simulink model "UR5_OpenLoop"  (R2023b)
settings: Solver=FixedStepAuto  StartTime=0.0  StopTime=t_max  FixedStep=dt_max  RelTol=1e-3
values from neighbouring files (symbols this model uses):
  dt_max = 0.01    [UR5_Details.m]    (also in mpc_script.m; smc.m)
(part 2 of 2)

== matlab function UR5_OpenLoop/UR5 Kineamatics and Dynamics ==
  data: q_1 input; q_2 input; q_3 input; T output; Jacobi output; M output; C output; G output; dq_1 input; dq_2 input; dq_3 input; g parameter
function [T,Jacobi, M,C,G]    = fwdKIN(q_1, q_2, q_3, dq_1, dq_2,dq_3, g)

% TRANSLATION MATRICES AND FORWARD KINEMATICS 
% (Position of EE from joint space)
T = [cos(q_1)*cos(q_2)*cos(q_3) - 1.0*cos(q_1)*sin(q_2)*sin(q_3), - 1.0*cos(q_1)*cos(q_2)*sin(q_3) - 1.0*cos(q_1)*cos(q_3)*sin(q_2),  1.0*sin(q_1), 0.425*cos(q_1)*cos(q_2);
cos(q_2)*cos(q_3)*sin(q_1) - 1.0*sin(q_1)*sin(q_2)*sin(q_3), - 1.0*cos(q_2)*sin(q_1)*sin(q_3) - 1.0*cos(q_3)*sin(q_1)*sin(q_2), -1.0*cos(q_1), 0.425*cos(q_2)*sin(q_1);
              1.0*cos(q_2)*sin(q_3) + 1.0*cos(q_3)*sin(q_2),                     1.0*cos(q_2)*cos(q_3) - 1.0*sin(q_2)*sin(q_3),             0, 0.425*sin(q_2) + 0.0892;
                                                          0,                                                                 0,             0,                     1.0];
 

% JACOBIAN MATRIX OF END EFFECTOR
Jacobi = [0.0265*cos(q_1) + 1.0*sin(q_1)*(0.2723*sin(q_2)*sin(q_3) - 1.0*cos(q_2)*(0.2723*cos(q_3) + 0.425)), -1.0*cos(q_1)*(0.2723*cos(q_2)*sin(q_3) + 1.0*sin(q_2)*(0.2723*cos(q_3) + 0.425)), -1.0*cos(q_1)*(0.2723*cos(q_2)*sin(q_3) + 0.2723*cos(q_3)*sin(q_2));
0.0265*sin(q_1) - 1.0*cos(q_1)*(0.2723*sin(q_2)*sin(q_3) - 1.0*cos(q_2)*(0.2723*cos(q_3) + 0.425)), -1.0*sin(q_1)*(0.2723*cos(q_2)*sin(q_3) + 1.0*sin(q_2)*(0.2723*cos(q_3) + 0.425)), -1.0*sin(q_1)*(0.2723*cos(q_2)*sin(q_3) + 0.2723*cos(q_3)*sin(q_2));
                                                                                                 0,                 1.0*cos(q_2)*(0.2723*cos(q_3) + 0.425) - 0.2723*sin(q_2)*sin(q_3),                 0.2723*cos(q_2)*cos(q_3) - 0.2723*sin(q_2)*sin(q_3);
                                                                                                 0,                                                                      1.0*sin(q_1),                                                        1.0*sin(q_1);
                                                                                                 0,                                                                     -1.0*cos(q_1),                                                       -1.0*cos(q_1);
                                                                                               1.0,                                                                                 0,                                                                   0];


%Robots Inertia (Mass Matrix)
M = [                                                 1.378e-5*cos(q_1)^2 + 0.0021*cos(q_2)^2 + 1.378e-5*sin(q_1)^2 + 0.0078*sin(q_2)^2 + (0.1134*cos(q_1) - 0.2125*cos(q_2)*sin(q_1))*(0.9514*cos(q_1) - 1.784*cos(q_2)*sin(q_1)) + (0.1134*sin(q_1) + 0.2125*cos(q_1)*cos(q_2))*(0.9514*sin(q_1) + 1.784*cos(q_1)*cos(q_2)) + (0.0265*cos(q_1) + 1.0*sin(q_1)*(0.2723*sin(q_2)*sin(q_3) - 1.0*cos(q_2)*(0.2723*cos(q_3) + 0.425)))*(0.06029*cos(q_1) + 2.275*sin(q_1)*(0.2723*sin(q_2)*sin(q_3) - 1.0*cos(q_2)*(0.2723*cos(q_3) + 0.425))) + (0.0265*sin(q_1) - 1.0*cos(q_1)*(0.2723*sin(q_2)*sin(q_3) - 1.0*cos(q_2)*(0.2723*cos(q_3) + 0.425)))*(0.06029*sin(q_1) - 2.275*cos(q_1)*(0.2723*sin(q_2)*sin(q_3) - 1.0*cos(q_2)*(0.2723*cos(q_3) + 0.425))) + 1.0*(1.0*cos(q_2)*cos(q_3) - 1.0*sin(q_2)*sin(q_3))*(0.0462*cos(q_2)*cos(q_3) - 0.0462*sin(q_2)*sin(q_3)) + 1.0*(1.0*cos(q_2)*sin(q_3) + 1.0*cos(q_3)*sin(q_2))*(0.0016*cos(q_2)*sin(q_3) + 0.0016*cos(q_3)*sin(q_2)) + 0.0084,                                                                                                                                                                                                                                                                                                                                                                                                                                                                                                                                                                          1.0*sin(q_1)*((0.0016*cos(q_2)*sin(q_3) + 0.0016*cos(q_3)*sin(q_2))*(cos(q_1)*cos(q_2)*cos(q_3) - 1.0*cos(q_1)*sin(q_2)*sin(q_3)) - 1.0*(0.0462*cos(q_2)*cos(q_3) - 0.0462*sin(q_2)*sin(q_3))*(1.0*cos(q_1)*cos(q_2)*sin(q_3) + 1.0*cos(q_1)*cos(q_3)*sin(q_2))) + 1.0*cos(q_1)*((0.0462*cos(q_2)*cos(q_3) - 0.0462*sin(q_2)*sin(q_3))*(1.0*cos(q_2)*sin(q_1)*sin(q_3) + 1.0*cos(q_3)*sin(q_1)*sin(q_2)) + (0.0016*cos(q_2)*sin(q_3) + 0.0016*cos(q_3)*sin(q_2))*(1.0*sin(q_1)*sin(q_2)*sin(q_3) - 1.0*cos(q_2)*cos(q_3)*sin(q_1))) - 0.2125*cos(q_1)*sin(q_2)*(0.9514*cos(q_1) - 1.784*cos(q_2)*sin(q_1)) - 0.2125*sin(q_1)*sin(q_2)*(0.9514*sin(q_1) + 1.784*cos(q_1)*cos(q_2)) - 1.0*cos(q_1)*(0.06029*cos(q_1) + 2.275*sin(q_1)*(0.2723*sin(q_2)*sin(q_3) - 1.0*cos(q_2)*(0.2723*cos(q_3) + 0.425)))*(0.2723*cos(q_2)*sin(q_3) + 1.0*sin(q_2)*(0.2723*cos(q_3) + 0.425)) - 1.0*sin(q_1)*(0.06029*sin(q_1) - 2.275*cos(q_1)*(0.2723*sin(q_2)*sin(q_3) - 1.0*cos(q_2)*(0.2723*cos(q_3) + 0.425)))*(0.2723*cos(q_2)*sin(q_3) + 1.0*sin(q_2)*(0.2723*cos(q_3) + 0.425)),                                                                                                                                                                                                                                                                                                                                                                                                                                                                                                                                                                                                                                                 1.0*sin(q_1)*((0.0016*cos(q_2)*sin(q_3) + 0.0016*cos(q_3)*sin(q_2))*(cos(q_1)*cos(q_2)*cos(q_3) - 1.0*cos(q_1)*sin(q_2)*sin(q_3)) - 1.0*(0.0462*cos(q_2)*cos(q_3) - 0.0462*sin(q_2)*sin(q_3))*(1.0*cos(q_1)*cos(q_2)*sin(q_3) + 1.0*cos(q_1)*cos(q_3)*sin(q_2))) + 1.0*cos(q_1)*((0.0462*cos(q_2)*cos(q_3) - 0.0462*sin(q_2)*sin(q_3))*(1.0*cos(q_2)*sin(q_1)*sin(q_3) + 1.0*cos(q_3)*sin(q_1)*sin(q_2)) + (0.0016*cos(q_2)*sin(q_3) + 0.0016*cos(q_3)*sin(q_2))*(1.0*sin(q_1)*sin(q_2)*sin(q_3) - 1.0*cos(q_2)*cos(q_3)*sin(q_1))) - 1.0*cos(q_1)*(0.2723*cos(q_2)*sin(q_3) + 0.2723*cos(q_3)*sin(q_2))*(0.06029*cos(q_1) + 2.275*sin(q_1)*(0.2723*sin(q_2)*sin(q_3) - 1.0*cos(q_2)*(0.2723*cos(q_3) + 0.425))) - 1.0*sin(q_1)*(0.2723*cos(q_2)*sin(q_3) + 0.2723*cos(q_3)*sin(q_2))*(0.06029*sin(q_1) - 2.275*cos(q_1)*(0.2723*sin(q_2)*sin(q_3) - 1.0*cos(q_2)*(0.2723*cos(q_3) + 0.425)));
1.0*(1.0*cos(q_2)*sin(q_3) + 1.0*cos(q_3)*sin(q_2))*(0.0016*cos(q_1)*(1.0*sin(q_1)*sin(q_2)*sin(q_3) - 1.0*cos(q_2)*cos(q_3)*sin(q_1)) + 0.0016*sin(q_1)*(cos(q_1)*cos(q_2)*cos(q_3) - 1.0*cos(q_1)*sin(q_2)*sin(q_3))) + 1.0*(1.0*cos(q_2)*cos(q_3) - 1.0*sin(q_2)*sin(q_3))*(0.0462*cos(q_1)*(1.0*cos(q_2)*sin(q_1)*sin(q_3) + 1.0*cos(q_3)*sin(q_1)*sin(q_2)) - 0.0462*sin(q_1)*(1.0*cos(q_1)*cos(q_2)*sin(q_3) + 1.0*cos(q_1)*cos(q_3)*sin(q_2))) - 1.784*cos(q_1)*sin(q_2)*(0.1134*cos(q_1) - 0.2125*cos(q_2)*sin(q_1)) - 1.784*sin(q_1)*sin(q_2)*(0.1134*sin(q_1) + 0.2125*cos(q_1)*cos(q_2)) - 2.275*cos(q_1)*(0.0265*cos(q_1) + 1.0*sin(q_1)*(0.2723*sin(q_2)*sin(q_3) - 1.0*cos(q_2)*(0.2723*cos(q_3) + 0.425)))*(0.2723*cos(q_2)*sin(q_3) + 1.0*sin(q_2)*(0.2723*cos(q_3) + 0.425)) - 2.275*sin(q_1)*(0.0265*sin(q_1) - 1.0*cos(q_1)*(0.2723*sin(q_2)*sin(q_3) - 1.0*cos(q_2)*(0.2723*cos(q_3) + 0.425)))*(0.2723*cos(q_2)*sin(q_3) + 1.0*sin(q_2)*(0.2723*cos(q_3) + 0.425)), 0.379*cos(q_2)^2 + 2.275*cos(q_1)^2*(0.2723*cos(q_2)*sin(q_3) + 1.0*sin(q_2)*(0.2723*cos(q_3) + 0.425))^2 + (0.2723*sin(q_2)*sin(q_3) - 1.0*cos(q_2)*(0.2723*cos(q_3) + 0.425))*(0.6195*sin(q_2)*sin(q_3) - 2.275*cos(q_2)*(0.2723*cos(q_3) + 0.425)) + 2.275*sin(q_1)^2*(0.2723*cos(q_2)*sin(q_3) + 1.0*sin(q_2)*(0.2723*cos(q_3) + 0.425))^2 + 1.0*cos(q_1)^2*(0.0021*cos(q_1)^2 + 0.0021*sin(q_1)^2) + 1.0*sin(q_1)^2*(0.0021*cos(q_1)^2 + 0.0021*sin(q_1)^2) + 0.379*cos(q_1)^2*sin(q_2)^2 + 1.0*sin(q_1)*(1.0*sin(q_1)*(0.0462*cos(q_1)^2 + 0.0462*sin(q_1)^2) - 1.0*(0.0462*cos(q_1)*(1.0*cos(q_2)*sin(q_1)*sin(q_3) + 1.0*cos(q_3)*sin(q_1)*sin(q_2)) - 0.0462*sin(q_1)*(1.0*cos(q_1)*cos(q_2)*sin(q_3) + 1.0*cos(q_1)*cos(q_3)*sin(q_2)))*(1.0*cos(q_1)*cos(q_2)*sin(q_3) + 1.0*cos(q_1)*cos(q_3)*sin(q_2)) + (cos(q_1)*cos(q_2)*cos(q_3) - 1.0*cos(q_1)*sin(q_2)*sin(q_3))*(0.0016*cos(q_1)*(1.0*sin(q_1)*sin(q_2)*sin(q_3) - 1.0*cos(q_2)*cos(q_3)*sin(q_1)) + 0.0016*sin(q_1)*(cos(q_1)*cos(q_2)*cos(q_3) - 1.0*cos(q_1)*sin(q_2)*sin(q_3)))) + 0.379*sin(q_1)^2*sin(q_2)^2 + 1.0*cos(q_1)*((1.0*sin(q_1)*sin(q_2)*sin(q_3) - 1.0*cos(q_2)*cos(q_3)*sin(q_1))*(0.0016*cos(q_1)*(1.0*sin(q_1)*sin(q_2)*sin(q_3) - 1.0*cos(q_2)*cos(q_3)*sin(q_1)) + 0.0016*sin(q_1)*(cos(q_1)*cos(q_2)*cos(q_3) - 1.0*cos(q_1)*sin(q_2)*sin(q_3))) + (0.0462*cos(q_1)*(1.0*cos(q_2)*sin(q_1)*sin(q_3) + 1.0*cos(q_3)*sin(q_1)*sin(q_2)) - 0.0462*sin(q_1)*(1.0*cos(q_1)*cos(q_2)*sin(q_3) + 1.0*cos(q_1)*cos(q_3)*sin(q_2)))*(1.0*cos(q_2)*sin(q_1)*sin(q_3) + 1.0*cos(q_3)*sin(q_1)*sin(q_2)) + 1.0*cos(q_1)*(0.0462*cos(q_1)^2 + 0.0462*sin(q_1)^2)), 1.0*sin(q_1)*(1.0*sin(q_1)*(0.0462*cos(q_1)^2 + 0.0462*sin(q_1)^2) - 1.0*(0.0462*cos(q_1)*(1.0*cos(q_2)*sin(q_1)*sin(q_3) + 1.0*cos(q_3)*sin(q_1)*sin(q_2)) - 0.0462*sin(q_1)*(1.0*cos(q_1)*cos(q_2)*sin(q_3) + 1.0*cos(q_1)*cos(q_3)*sin(q_2)))*(1.0*cos(q_1)*cos(q_2)*sin(q_3) + 1.0*cos(q_1)*cos(q_3)*sin(q_2)) + (cos(q_1)*cos(q_2)*cos(q_3) - 1.0*cos(q_1)*sin(q_2)*sin(q_3))*(0.0016*cos(q_1)*(1.0*sin(q_1)*sin(q_2)*sin(q_3) - 1.0*cos(q_2)*cos(q_3)*sin(q_1)) + 0.0016*sin(q_1)*(cos(q_1)*cos(q_2)*cos(q_3) - 1.0*cos(q_1)*sin(q_2)*sin(q_3)))) - 1.0*(0.2723*cos(q_2)*cos(q_3) - 0.2723*sin(q_2)*sin(q_3))*(0.6195*sin(q_2)*sin(q_3) - 2.275*cos(q_2)*(0.2723*cos(q_3) + 0.425)) + 1.0*cos(q_1)*((1.0*sin(q_1)*sin(q_2)*sin(q_3) - 1.0*cos(q_2)*cos(q_3)*sin(q_1))*(0.0016*cos(q_1)*(1.0*sin(q_1)*sin(q_2)*sin(q_3) - 1.0*cos(q_2)*cos(q_3)*sin(q_1)) + 0.0016*sin(q_1)*(cos(q_1)*cos(q_2)*cos(q_3) - 1.0*cos(q_1)*sin(q_2)*sin(q_3))) + (0.0462*cos(q_1)*(1.0*cos(q_2)*sin(q_1)*sin(q_3) + 1.0*cos(q_3)*sin(q_1)*sin(q_2)) - 0.0462*sin(q_1)*(1.0*cos(q_1)*cos(q_2)*sin(q_3) + 1.0*cos(q_1)*cos(q_3)*sin(q_2)))*(1.0*cos(q_2)*sin(q_1)*sin(q_3) + 1.0*cos(q_3)*sin(q_1)*sin(q_2)) + 1.0*cos(q_1)*(0.0462*cos(q_1)^2 + 0.0462*sin(q_1)^2)) + 2.275*cos(q_1)^2*(0.2723*cos(q_2)*sin(q_3) + 0.2723*cos(q_3)*sin(q_2))*(0.2723*cos(q_2)*sin(q_3) + 1.0*sin(q_2)*(0.2723*cos(q_3) + 0.425)) + 2.275*sin(q_1)^2*(0.2723*cos(q_2)*sin(q_3) + 0.2723*cos(q_3)*sin(q_2))*(0.2723*cos(q_2)*sin(q_3) + 1.0*sin(q_2)*(0.2723*cos(q_3) + 0.425));
                                                                                                                                                                          1.0*(1.0*cos(q_2)*sin(q_3) + 1.0*cos(q_3)*sin(q_2))*(0.0016*cos(q_1)*(1.0*sin(q_1)*sin(q_2)*sin(q_3) - 1.0*cos(q_2)*cos(q_3)*sin(q_1)) + 0.0016*sin(q_1)*(cos(q_1)*cos(q_2)*cos(q_3) - 1.0*cos(q_1)*sin(q_2)*sin(q_3))) + 1.0*(1.0*cos(q_2)*cos(q_3) - 1.0*sin(q_2)*sin(q_3))*(0.0462*cos(q_1)*(1.0*cos(q_2)*sin(q_1)*sin(q_3) + 1.0*cos(q_3)*sin(q_1)*sin(q_2)) - 0.0462*sin(q_1)*(1.0*cos(q_1)*cos(q_2)*sin(q_3) + 1.0*cos(q_1)*cos(q_3)*sin(q_2))) - 2.275*cos(q_1)*(0.0265*cos(q_1) + 1.0*sin(q_1)*(0.2723*sin(q_2)*sin(q_3) - 1.0*cos(q_2)*(0.2723*cos(q_3) + 0.425)))*(0.2723*cos(q_2)*sin(q_3) + 0.2723*cos(q_3)*sin(q_2)) - 2.275*sin(q_1)*(0.0265*sin(q_1) - 1.0*cos(q_1)*(0.2723*sin(q_2)*sin(q_3) - 1.0*cos(q_2)*(0.2723*cos(q_3) + 0.425)))*(0.2723*cos(q_2)*sin(q_3) + 0.2723*cos(q_3)*sin(q_2)),                                                                                                      1.0*sin(q_1)*(1.0*sin(q_1)*(0.0462*cos(q_1)^2 + 0.0462*sin(q_1)^2) - 1.0*(0.0462*cos(q_1)*(1.0*cos(q_2)*sin(q_1)*sin(q_3) + 1.0*cos(q_3)*sin(q_1)*sin(q_2)) - 0.0462*sin(q_1)*(1.0*cos(q_1)*cos(q_2)*sin(q_3) + 1.0*cos(q_1)*cos(q_3)*sin(q_2)))*(1.0*cos(q_1)*cos(q_2)*sin(q_3) + 1.0*cos(q_1)*cos(q_3)*sin(q_2)) + (cos(q_1)*cos(q_2)*cos(q_3) - 1.0*cos(q_1)*sin(q_2)*sin(q_3))*(0.0016*cos(q_1)*(1.0*sin(q_1)*sin(q_2)*sin(q_3) - 1.0*cos(q_2)*cos(q_3)*sin(q_1)) + 0.0016*sin(q_1)*(cos(q_1)*cos(q_2)*cos(q_3) - 1.0*cos(q_1)*sin(q_2)*sin(q_3)))) - 1.0*(0.6195*cos(q_2)*cos(q_3) - 0.6195*sin(q_2)*sin(q_3))*(0.2723*sin(q_2)*sin(q_3) - 1.0*cos(q_2)*(0.2723*cos(q_3) + 0.425)) + 1.0*cos(q_1)*((1.0*sin(q_1)*sin(q_2)*sin(q_3) - 1.0*cos(q_2)*cos(q_3)*sin(q_1))*(0.0016*cos(q_1)*(1.0*sin(q_1)*sin(q_2)*sin(q_3) - 1.0*cos(q_2)*cos(q_3)*sin(q_1)) + 0.0016*sin(q_1)*(cos(q_1)*cos(q_2)*cos(q_3) - 1.0*cos(q_1)*sin(q_2)*sin(q_3))) + (0.0462*cos(q_1)*(1.0*cos(q_2)*sin(q_1)*sin(q_3) + 1.0*cos(q_3)*sin(q_1)*sin(q_2)) - 0.0462*sin(q_1)*(1.0*cos(q_1)*cos(q_2)*sin(q_3) + 1.0*cos(q_1)*cos(q_3)*sin(q_2)))*(1.0*cos(q_2)*sin(q_1)*sin(q_3) + 1.0*cos(q_3)*sin(q_1)*sin(q_2)) + 1.0*cos(q_1)*(0.0462*cos(q_1)^2 + 0.0462*sin(q_1)^2)) + 2.275*cos(q_1)^2*(0.2723*cos(q_2)*sin(q_3) + 0.2723*cos(q_3)*sin(q_2))*(0.2723*cos(q_2)*sin(q_3) + 1.0*sin(q_2)*(0.2723*cos(q_3) + 0.425)) + 2.275*sin(q_1)^2*(0.2723*cos(q_2)*sin(q_3) + 0.2723*cos(q_3)*sin(q_2))*(0.2723*cos(q_2)*sin(q_3) + 1.0*sin(q_2)*(0.2723*cos(q_3) + 0.425)),                                                                                                                                                         2.275*cos(q_1)^2*(0.2723*cos(q_2)*sin(q_3) + 0.2723*cos(q_3)*sin(q_2))^2 + 2.275*sin(q_1)^2*(0.2723*cos(q_2)*sin(q_3) + 0.2723*cos(q_3)*sin(q_2))^2 + (0.2723*cos(q_2)*cos(q_3) - 0.2723*sin(q_2)*sin(q_3))*(0.6195*cos(q_2)*cos(q_3) - 0.6195*sin(q_2)*sin(q_3)) + 1.0*sin(q_1)*(1.0*sin(q_1)*(0.0462*cos(q_1)^2 + 0.0462*sin(q_1)^2) - 1.0*(0.0462*cos(q_1)*(1.0*cos(q_2)*sin(q_1)*sin(q_3) + 1.0*cos(q_3)*sin(q_1)*sin(q_2)) - 0.0462*sin(q_1)*(1.0*cos(q_1)*cos(q_2)*sin(q_3) + 1.0*cos(q_1)*cos(q_3)*sin(q_2)))*(1.0*cos(q_1)*cos(q_2)*sin(q_3) + 1.0*cos(q_1)*cos(q_3)*sin(q_2)) + (cos(q_1)*cos(q_2)*cos(q_3) - 1.0*cos(q_1)*sin(q_2)*sin(q_3))*(0.0016*cos(q_1)*(1.0*sin(q_1)*sin(q_2)*sin(q_3) - 1.0*cos(q_2)*cos(q_3)*sin(q_1)) + 0.0016*sin(q_1)*(cos(q_1)*cos(q_2)*cos(q_3) - 1.0*cos(q_1)*sin(q_2)*sin(q_3)))) + 1.0*cos(q_1)*((1.0*sin(q_1)*sin(q_2)*sin(q_3) - 1.0*cos(q_2)*cos(q_3)*sin(q_1))*(0.0016*cos(q_1)*(1.0*sin(q_1)*sin(q_2)*sin(q_3) - 1.0*cos(q_2)*cos(q_3)*sin(q_1)) + 0.0016*sin(q_1)*(cos(q_1)*cos(q_2)*cos(q_3) - 1.0*cos(q_1)*sin(q_2)*sin(q_3))) + (0.0462*cos(q_1)*(1.0*cos(q_2)*sin(q_1)*sin(q_3) + 1.0*cos(q_3)*sin(q_1)*sin(q_2)) - 0.0462*sin(q_1)*(1.0*cos(q_1)*cos(q_2)*sin(q_3) + 1.0*cos(q_1)*cos(q_3)*sin(q_2)))*(1.0*cos(q_2)*sin(q_1)*sin(q_3) + 1.0*cos(q_3)*sin(q_1)*sin(q_2)) + 1.0*cos(q_1)*(0.0462*cos(q_1)^2 + 0.0462*sin(q_1)^2))];
 

% CORIOLIS and CENTRIFUGAL MATRIX
C = [                                                                                                                                                                                                                                                                                                                                                                                                                                                                                                                                                                                                                                                                                                                                                                                                                                                                                                                                                                                                                                                                                                                                                                                                                                                                                                                                                                                                                                                                                                                                                                                                                                                                                                                                                                                                                                                                                                                                                                                                                                                                                                                                                                                                                                                                                                                                                                   0.5*dq_2*(1.0*sin(q_1)*(1.0*(0.0462*cos(q_2)*cos(q_3) - 0.0462*sin(q_2)*sin(q_3))*(1.0*cos(q_2)*sin(q_1)*sin(q_3) + 1.0*cos(q_3)*sin(q_1)*sin(q_2)) + (0.0016*cos(q_2)*sin(q_3) + 0.0016*cos(q_3)*sin(q_2))*(1.0*sin(q_1)*sin(q_2)*sin(q_3) - 1.0*cos(q_2)*cos(q_3)*sin(q_1))) + 0.0114*cos(q_2)*sin(q_2) - 1.0*(1.0*cos(q_2)*sin(q_3) + 1.0*cos(q_3)*sin(q_2))*(0.0016*cos(q_1)*(cos(q_1)*cos(q_2)*cos(q_3) - 1.0*cos(q_1)*sin(q_2)*sin(q_3)) - 0.0016*cos(q_1)*(1.0*cos(q_1)*cos(q_2)*cos(q_3) - 1.0*cos(q_1)*sin(q_2)*sin(q_3))) + 1.0*cos(q_1)*((0.0016*cos(q_2)*sin(q_3) + 0.0016*cos(q_3)*sin(q_2))*(cos(q_1)*cos(q_2)*cos(q_3) - 1.0*cos(q_1)*sin(q_2)*sin(q_3)) - 1.0*(0.0462*cos(q_2)*cos(q_3) - 0.0462*sin(q_2)*sin(q_3))*(1.0*cos(q_1)*cos(q_2)*sin(q_3) + 1.0*cos(q_1)*cos(q_3)*sin(q_2))) + 1.0*cos(q_1)*((0.0462*cos(q_2)*cos(q_3) - 0.0462*sin(q_2)*sin(q_3))*(1.0*cos(q_1)*cos(q_2)*sin(q_3) + 1.0*cos(q_1)*cos(q_3)*sin(q_2)) - 1.0*(0.0016*cos(q_2)*sin(q_3) + 0.0016*cos(q_3)*sin(q_2))*(1.0*cos(q_1)*cos(q_2)*cos(q_3) - 1.0*cos(q_1)*sin(q_2)*sin(q_3))) - 1.0*(1.0*cos(q_2)*cos(q_3) - 1.0*sin(q_2)*sin(q_3))*(0.0462*cos(q_2)*sin(q_3) + 0.0462*cos(q_3)*sin(q_2)) - 1.0*(1.0*cos(q_2)*sin(q_3) + 1.0*cos(q_3)*sin(q_2))*(0.0462*cos(q_2)*cos(q_3) - 0.0462*sin(q_2)*sin(q_3)) - 1.0*sin(q_1)*((0.0462*cos(q_2)*cos(q_3) - 0.0462*sin(q_2)*sin(q_3))*(1.0*cos(q_2)*sin(q_1)*sin(q_3) + 1.0*cos(q_3)*sin(q_1)*sin(q_2)) + (0.0016*cos(q_2)*sin(q_3) + 0.0016*cos(q_3)*sin(q_2))*(1.0*sin(q_1)*sin(q_2)*sin(q_3) - 1.0*cos(q_2)*cos(q_3)*sin(q_1))) + 1.0*(1.0*cos(q_2)*cos(q_3) - 1.0*sin(q_2)*sin(q_3))*(0.0016*cos(q_2)*sin(q_3) + 0.0016*cos(q_3)*sin(q_2)) + 1.0*(1.0*cos(q_2)*sin(q_3) + 1.0*cos(q_3)*sin(q_2))*(0.0016*cos(q_2)*cos(q_3) - 0.0016*sin(q_2)*sin(q_3)) - 1.784*cos(q_1)*sin(q_2)*(0.1134*sin(q_1) + 0.2125*cos(q_1)*cos(q_2)) - 0.2125*cos(q_1)*sin(q_2)*(0.9514*sin(q_1) + 1.784*cos(q_1)*cos(q_2)) + 1.784*sin(q_1)*sin(q_2)*(0.1134*cos(q_1) - 0.2125*cos(q_2)*sin(q_1)) + 0.2125*sin(q_1)*sin(q_2)*(0.9514*cos(q_1) - 1.784*cos(q_2)*sin(q_1)) - 2.275*cos(q_1)*(0.0265*sin(q_1) - 1.0*cos(q_1)*(0.2723*sin(q_2)*sin(q_3) - 1.0*cos(q_2)*(0.2723*cos(q_3) + 0.425)))*(0.2723*cos(q_2)*sin(q_3) + 1.0*sin(q_2)*(0.2723*cos(q_3) + 0.425)) + 2.275*sin(q_1)*(0.0265*cos(q_1) + 1.0*sin(q_1)*(0.2723*sin(q_2)*sin(q_3) - 1.0*cos(q_2)*(0.2723*cos(q_3) + 0.425)))*(0.2723*cos(q_2)*sin(q_3) + 1.0*sin(q_2)*(0.2723*cos(q_3) + 0.425)) - 1.0*cos(q_1)*(0.06029*sin(q_1) - 2.275*cos(q_1)*(0.2723*sin(q_2)*sin(q_3) - 1.0*cos(q_2)*(0.2723*cos(q_3) + 0.425)))*(0.2723*cos(q_2)*sin(q_3) + 1.0*sin(q_2)*(0.2723*cos(q_3) + 0.425)) + 1.0*sin(q_1)*(0.06029*cos(q_1) + 2.275*sin(q_1)*(0.2723*sin(q_2)*sin(q_3) - 1.0*cos(q_2)*(0.2723*cos(q_3) + 0.425)))*(0.2723*cos(q_2)*sin(q_3) + 1.0*sin(q_2)*(0.2723*cos(q_3) + 0.425))) + 0.5*dq_3*(1.0*sin(q_1)*(1.0*(0.0462*cos(q_2)*cos(q_3) - 0.0462*sin(q_2)*sin(q_3))*(1.0*cos(q_2)*sin(q_1)*sin(q_3) + 1.0*cos(q_3)*sin(q_1)*sin(q_2)) + (0.0016*cos(q_2)*sin(q_3) + 0.0016*cos(q_3)*sin(q_2))*(1.0*sin(q_1)*sin(q_2)*sin(q_3) - 1.0*cos(q_2)*cos(q_3)*sin(q_1))) - 1.0*(1.0*cos(q_2)*sin(q_3) + 1.0*cos(q_3)*sin(q_2))*(0.0016*cos(q_1)*(cos(q_1)*cos(q_2)*cos(q_3) - 1.0*cos(q_1)*sin(q_2)*sin(q_3)) - 0.0016*cos(q_1)*(1.0*cos(q_1)*cos(q_2)*cos(q_3) - 1.0*cos(q_1)*sin(q_2)*sin(q_3))) + 1.0*cos(q_1)*((0.0016*cos(q_2)*sin(q_3) + 0.0016*cos(q_3)*sin(q_2))*(cos(q_1)*cos(q_2)*cos(q_3) - 1.0*cos(q_1)*sin(q_2)*sin(q_3)) - 1.0*(0.0462*cos(q_2)*cos(q_3) - 0.0462*sin(q_2)*sin(q_3))*(1.0*cos(q_1)*cos(q_2)*sin(q_3) + 1.0*cos(q_1)*cos(q_3)*sin(q_2))) + 1.0*cos(q_1)*((0.0462*cos(q_2)*cos(q_3) - 0.0462*sin(q_2)*sin(q_3))*(1.0*cos(q_1)*cos(q_2)*sin(q_3) + 1.0*cos(q_1)*cos(q_3)*sin(q_2)) - 1.0*(0.0016*cos(q_2)*sin(q_3) + 0.0016*cos(q_3)*sin(q_2))*(1.0*cos(q_1)*cos(q_2)*cos(q_3) - 1.0*cos(q_1)*sin(q_2)*sin(q_3))) - 1.0*(1.0*cos(q_2)*cos(q_3) - 1.0*sin(q_2)*sin(q_3))*(0.0462*cos(q_2)*sin(q_3) + 0.0462*cos(q_3)*sin(q_2)) - 1.0*(1.0*cos(q_2)*sin(q_3) + 1.0*cos(q_3)*sin(q_2))*(0.0462*cos(q_2)*cos(q_3) - 0.0462*sin(q_2)*sin(q_3)) - 1.0*sin(q_1)*((0.0462*cos(q_2)*cos(q_3) - 0.0462*sin(q_2)*sin(q_3))*(1.0*cos(q_2)*sin(q_1)*sin(q_3) + 1.0*cos(q_3)*sin(q_1)*sin(q_2)) + (0.0016*cos(q_2)*sin(q_3) + 0.0016*cos(q_3)*sin(q_2))*(1.0*sin(q_1)*sin(q_2)*sin(q_3) - 1.0*cos(q_2)*cos(q_3)*sin(q_1))) + 1.0*(1.0*cos(q_2)*cos(q_3) - 1.0*sin(q_2)*sin(q_3))*(0.0016*cos(q_2)*sin(q_3) + 0.0016*cos(q_3)*sin(q_2)) + 1.0*(1.0*cos(q_2)*sin(q_3) + 1.0*cos(q_3)*sin(q_2))*(0.0016*cos(q_2)*cos(q_3) - 0.0016*sin(q_2)*sin(q_3)) - 2.275*cos(q_1)*(0.0265*sin(q_1) - 1.0*cos(q_1)*(0.2723*sin(q_2)*sin(q_3) - 1.0*cos(q_2)*(0.2723*cos(q_3) + 0.425)))*(0.2723*cos(q_2)*sin(q_3) + 0.2723*cos(q_3)*sin(q_2)) + 2.275*sin(q_1)*(0.0265*cos(q_1) + 1.0*sin(q_1)*(0.2723*sin(q_2)*sin(q_3) - 1.0*cos(q_2)*(0.2723*cos(q_3) + 0.425)))*(0.2723*cos(q_2)*sin(q_3) + 0.2723*cos(q_3)*sin(q_2)) - 1.0*cos(q_1)*(0.2723*cos(q_2)*sin(q_3) + 0.2723*cos(q_3)*sin(q_2))*(0.06029*sin(q_1) - 2.275*cos(q_1)*(0.2723*sin(q_2)*sin(q_3) - 1.0*cos(q_2)*(0.2723*cos(q_3) + 0.425))) + 1.0*sin(q_1)*(0.2723*cos(q_2)*sin(q_3) + 0.2723*cos(q_3)*sin(q_2))*(0.06029*cos(q_1) + 2.275*sin(q_1)*(0.2723*sin(q_2)*sin(q_3) - 1.0*cos(q_2)*(0.2723*cos(q_3) + 0.425)))),                                                                                                                                                                                                                                                                                                                                                                                                                                                                                                                                                                                                                                                                                                                                                                                                                                                                                                                                                                                                                                                                                                                                                                                                                                                                                                                                                                                                                                                                                                                                                                                                                                                                                                                                                                                                                                                                                                                                                                                                                                                                                                                                                             0.5*dq_1*(0.0114*cos(q_2)*sin(q_2) - 1.0*(1.0*cos(q_2)*cos(q_3) - 1.0*sin(q_2)*sin(q_3))*(0.0462*cos(q_2)*sin(q_3) + 0.0462*cos(q_3)*sin(q_2)) - 1.0*(1.0*cos(q_2)*sin(q_3) + 1.0*cos(q_3)*sin(q_2))*(0.0462*cos(q_2)*cos(q_3) - 0.0462*sin(q_2)*sin(q_3)) + 1.0*(1.0*cos(q_2)*cos(q_3) - 1.0*sin(q_2)*sin(q_3))*(0.0016*cos(q_2)*sin(q_3) + 0.0016*cos(q_3)*sin(q_2)) + 1.0*(1.0*cos(q_2)*sin(q_3) + 1.0*cos(q_3)*sin(q_2))*(0.0016*cos(q_2)*cos(q_3) - 0.0016*sin(q_2)*sin(q_3)) - 1.784*cos(q_1)*sin(q_2)*(0.1134*sin(q_1) + 0.2125*cos(q_1)*cos(q_2)) - 0.2125*cos(q_1)*sin(q_2)*(0.9514*sin(q_1) + 1.784*cos(q_1)*cos(q_2)) + 1.784*sin(q_1)*sin(q_2)*(0.1134*cos(q_1) - 0.2125*cos(q_2)*sin(q_1)) + 0.2125*sin(q_1)*sin(q_2)*(0.9514*cos(q_1) - 1.784*cos(q_2)*sin(q_1)) - 2.275*cos(q_1)*(0.0265*sin(q_1) - 1.0*cos(q_1)*(0.2723*sin(q_2)*sin(q_3) - 1.0*cos(q_2)*(0.2723*cos(q_3) + 0.425)))*(0.2723*cos(q_2)*sin(q_3) + 1.0*sin(q_2)*(0.2723*cos(q_3) + 0.425)) + 2.275*sin(q_1)*(0.0265*cos(q_1) + 1.0*sin(q_1)*(0.2723*sin(q_2)*sin(q_3) - 1.0*cos(q_2)*(0.2723*cos(q_3) + 0.425)))*(0.2723*cos(q_2)*sin(q_3) + 1.0*sin(q_2)*(0.2723*cos(q_3) + 0.425)) - 1.0*cos(q_1)*(0.06029*sin(q_1) - 2.275*cos(q_1)*(0.2723*sin(q_2)*sin(q_3) - 1.0*cos(q_2)*(0.2723*cos(q_3) + 0.425)))*(0.2723*cos(q_2)*sin(q_3) + 1.0*sin(q_2)*(0.2723*cos(q_3) + 0.425)) + 1.0*sin(q_1)*(0.06029*cos(q_1) + 2.275*sin(q_1)*(0.2723*sin(q_2)*sin(q_3) - 1.0*cos(q_2)*(0.2723*cos(q_3) + 0.425)))*(0.2723*cos(q_2)*sin(q_3) + 1.0*sin(q_2)*(0.2723*cos(q_3) + 0.425))) - 0.5*dq_2*(1.0*sin(q_1)*((1.0*sin(q_1)*sin(q_2)*sin(q_3) - 1.0*cos(q_2)*cos(q_3)*sin(q_1))*(0.0016*cos(q_1)*(1.0*sin(q_1)*sin(q_2)*sin(q_3) - 1.0*cos(q_2)*cos(q_3)*sin(q_1)) + 0.0016*sin(q_1)*(cos(q_1)*cos(q_2)*cos(q_3) - 1.0*cos(q_1)*sin(q_2)*sin(q_3))) + 1.0*(0.0462*cos(q_1)*(1.0*cos(q_2)*sin(q_1)*sin(q_3) + 1.0*cos(q_3)*sin(q_1)*sin(q_2)) - 0.0462*sin(q_1)*(1.0*cos(q_1)*cos(q_2)*sin(q_3) + 1.0*cos(q_1)*cos(q_3)*sin(q_2)))*(1.0*cos(q_2)*sin(q_1)*sin(q_3) + 1.0*cos(q_3)*sin(q_1)*sin(q_2)) + 1.0*cos(q_1)*(0.0462*cos(q_1)^2 + 0.0462*sin(q_1)^2) + 1.0*(cos(q_1)*cos(q_2)*cos(q_3) - 1.0*cos(q_1)*sin(q_2)*sin(q_3))*(0.0016*cos(q_1)*(cos(q_1)*cos(q_2)*cos(q_3) - 1.0*cos(q_1)*sin(q_2)*sin(q_3)) - 0.0016*cos(q_1)*(1.0*cos(q_1)*cos(q_2)*cos(q_3) - 1.0*cos(q_1)*sin(q_2)*sin(q_3)))) - 1.0*sin(q_1)*((1.0*sin(q_1)*sin(q_2)*sin(q_3) - 1.0*cos(q_2)*cos(q_3)*sin(q_1))*(0.0016*cos(q_1)*(1.0*sin(q_1)*sin(q_2)*sin(q_3) - 1.0*cos(q_2)*cos(q_3)*sin(q_1)) + 0.0016*sin(q_1)*(cos(q_1)*cos(q_2)*cos(q_3) - 1.0*cos(q_1)*sin(q_2)*sin(q_3))) + (0.0462*cos(q_1)*(1.0*cos(q_2)*sin(q_1)*sin(q_3) + 1.0*cos(q_3)*sin(q_1)*sin(q_2)) - 0.0462*sin(q_1)*(1.0*cos(q_1)*cos(q_2)*sin(q_3) + 1.0*cos(q_1)*cos(q_3)*sin(q_2)))*(1.0*cos(q_2)*sin(q_1)*sin(q_3) + 1.0*cos(q_3)*sin(q_1)*sin(q_2)) + 1.0*cos(q_1)*(0.0462*cos(q_1)^2 + 0.0462*sin(q_1)^2)) + 1.0*cos(q_1)*((0.0016*cos(q_1)*(cos(q_1)*cos(q_2)*cos(q_3) - 1.0*cos(q_1)*sin(q_2)*sin(q_3)) - 0.0016*cos(q_1)*(1.0*cos(q_1)*cos(q_2)*cos(q_3) - 1.0*cos(q_1)*sin(q_2)*sin(q_3)))*(1.0*sin(q_1)*sin(q_2)*sin(q_3) - 1.0*cos(q_2)*cos(q_3)*sin(q_1)) - 1.0*(1.0*cos(q_1)*cos(q_2)*cos(q_3) - 1.0*cos(q_1)*sin(q_2)*sin(q_3))*(0.0016*cos(q_1)*(1.0*sin(q_1)*sin(q_2)*sin(q_3) - 1.0*cos(q_2)*cos(q_3)*sin(q_1)) + 0.0016*sin(q_1)*(cos(q_1)*cos(q_2)*cos(q_3) - 1.0*cos(q_1)*sin(q_2)*sin(q_3))) + 1.0*(0.0462*cos(q_1)*(1.0*cos(q_2)*sin(q_1)*sin(q_3) + 1.0*cos(q_3)*sin(q_1)*sin(q_2)) - 0.0462*sin(q_1)*(1.0*cos(q_1)*cos(q_2)*sin(q_3) + 1.0*cos(q_1)*cos(q_3)*sin(q_2)))*(1.0*cos(q_1)*cos(q_2)*sin(q_3) + 1.0*cos(q_1)*cos(q_3)*sin(q_2)) - 1.0*sin(q_1)*(0.0462*cos(q_1)^2 + 0.0462*sin(q_1)^2)) + 2.0*cos(q_1)*((0.0462*cos(q_2)*cos(q_3) - 0.0462*sin(q_2)*sin(q_3))*(1.0*sin(q_1)*sin(q_2)*sin(q_3) - 1.0*cos(q_2)*cos(q_3)*sin(q_1)) + (0.0462*cos(q_2)*sin(q_3) + 0.0462*cos(q_3)*sin(q_2))*(1.0*cos(q_2)*sin(q_1)*sin(q_3) + 1.0*cos(q_3)*sin(q_1)*sin(q_2)) - 1.0*(0.0016*cos(q_2)*cos(q_3) - 0.0016*sin(q_2)*sin(q_3))*(1.0*sin(q_1)*sin(q_2)*sin(q_3) - 1.0*cos(q_2)*cos(q_3)*sin(q_1)) - 1.0*(0.0016*cos(q_2)*sin(q_3) + 0.0016*cos(q_3)*sin(q_2))*(1.0*cos(q_2)*sin(q_1)*sin(q_3) + 1.0*cos(q_3)*sin(q_1)*sin(q_2))) - 2.0*sin(q_1)*((0.0016*cos(q_2)*cos(q_3) - 0.0016*sin(q_2)*sin(q_3))*(cos(q_1)*cos(q_2)*cos(q_3) - 1.0*cos(q_1)*sin(q_2)*sin(q_3)) - 1.0*(0.0016*cos(q_2)*sin(q_3) + 0.0016*cos(q_3)*sin(q_2))*(1.0*cos(q_1)*cos(q_2)*sin(q_3) + cos(q_1)*cos(q_3)*sin(q_2)) - 1.0*(0.0462*cos(q_2)*cos(q_3) - 0.0462*sin(q_2)*sin(q_3))*(1.0*cos(q_1)*cos(q_2)*cos(q_3) - 1.0*cos(q_1)*sin(q_2)*sin(q_3)) + 1.0*(0.0462*cos(q_2)*sin(q_3) + 0.0462*cos(q_3)*sin(q_2))*(1.0*cos(q_1)*cos(q_2)*sin(q_3) + 1.0*cos(q_1)*cos(q_3)*sin(q_2))) + 1.0*cos(q_1)*(1.0*sin(q_1)*(0.0462*cos(q_1)^2 + 0.0462*sin(q_1)^2) - 1.0*(0.0462*cos(q_1)*(1.0*cos(q_2)*sin(q_1)*sin(q_3) + 1.0*cos(q_3)*sin(q_1)*sin(q_2)) - 0.0462*sin(q_1)*(1.0*cos(q_1)*cos(q_2)*sin(q_3) + 1.0*cos(q_1)*cos(q_3)*sin(q_2)))*(1.0*cos(q_1)*cos(q_2)*sin(q_3) + 1.0*cos(q_1)*cos(q_3)*sin(q_2)) + (cos(q_1)*cos(q_2)*cos(q_3) - 1.0*cos(q_1)*sin(q_2)*sin(q_3))*(0.0016*cos(q_1)*(1.0*sin(q_1)*sin(q_2)*sin(q_3) - 1.0*cos(q_2)*cos(q_3)*sin(q_1)) + 0.0016*sin(q_1)*(cos(q_1)*cos(q_2)*cos(q_3) - 1.0*cos(q_1)*sin(q_2)*sin(q_3)))) + 0.425*cos(q_1)*cos(q_2)*(0.9514*cos(q_1) - 1.784*cos(q_2)*sin(q_1)) + 0.425*cos(q_2)*sin(q_1)*(0.9514*sin(q_1) + 1.784*cos(q_1)*cos(q_2)) - 2.0*cos(q_1)*(0.06029*cos(q_1) + 2.275*sin(q_1)*(0.2723*sin(q_2)*sin(q_3) - 1.0*cos(q_2)*(0.2723*cos(q_3) + 0.425)))*(0.2723*sin(q_2)*sin(q_3) - 1.0*cos(q_2)*(0.2723*cos(q_3) + 0.425)) - 2.0*sin(q_1)*(0.06029*sin(q_1) - 2.275*cos(q_1)*(0.2723*sin(q_2)*sin(q_3) - 1.0*cos(q_2)*(0.2723*cos(q_3) + 0.425)))*(0.2723*sin(q_2)*sin(q_3) - 1.0*cos(q_2)*(0.2723*cos(q_3) + 0.425))) - 0.5*dq_3*(1.0*sin(q_1)*((1.0*sin(q_1)*sin(q_2)*sin(q_3) - 1.0*cos(q_2)*cos(q_3)*sin(q_1))*(0.0016*cos(q_1)*(1.0*sin(q_1)*sin(q_2)*sin(q_3) - 1.0*cos(q_2)*cos(q_3)*sin(q_1)) + 0.0016*sin(q_1)*(cos(q_1)*cos(q_2)*cos(q_3) - 1.0*cos(q_1)*sin(q_2)*sin(q_3))) + 1.0*(0.0462*cos(q_1)*(1.0*cos(q_2)*sin(q_1)*sin(q_3) + 1.0*cos(q_3)*sin(q_1)*sin(q_2)) - 0.0462*sin(q_1)*(1.0*cos(q_1)*cos(q_2)*sin(q_3) + 1.0*cos(q_1)*cos(q_3)*sin(q_2)))*(1.0*cos(q_2)*sin(q_1)*sin(q_3) + 1.0*cos(q_3)*sin(q_1)*sin(q_2)) + 1.0*cos(q_1)*(0.0462*cos(q_1)^2 + 0.0462*sin(q_1)^2) + 1.0*(cos(q_1)*cos(q_2)*cos(q_3) - 1.0*cos(q_1)*sin(q_2)*sin(q_3))*(0.0016*cos(q_1)*(cos(q_1)*cos(q_2)*cos(q_3) - 1.0*cos(q_1)*sin(q_2)*sin(q_3)) - 0.0016*cos(q_1)*(1.0*cos(q_1)*cos(q_2)*cos(q_3) - 1.0*cos(q_1)*sin(q_2)*sin(q_3)))) - 1.0*sin(q_1)*((1.0*sin(q_1)*sin(q_2)*sin(q_3) - 1.0*cos(q_2)*cos(q_3)*sin(q_1))*(0.0016*cos(q_1)*(1.0*sin(q_1)*sin(q_2)*sin(q_3) - 1.0*cos(q_2)*cos(q_3)*sin(q_1)) + 0.0016*sin(q_1)*(cos(q_1)*cos(q_2)*cos(q_3) - 1.0*cos(q_1)*sin(q_2)*sin(q_3))) + (0.0462*cos(q_1)*(1.0*cos(q_2)*sin(q_1)*sin(q_3) + 1.0*cos(q_3)*sin(q_1)*sin(q_2)) - 0.0462*sin(q_1)*(1.0*cos(q_1)*cos(q_2)*sin(q_3) + 1.0*cos(q_1)*cos(q_3)*sin(q_2)))*(1.0*cos(q_2)*sin(q_1)*sin(q_3) + 1.0*cos(q_3)*sin(q_1)*sin(q_2)) + 1.0*cos(q_1)*(0.0462*cos(q_1)^2 + 0.0462*sin(q_1)^2)) + 1.0*cos(q_1)*((0.0016*cos(q_1)*(cos(q_1)*cos(q_2)*cos(q_3) - 1.0*cos(q_1)*sin(q_2)*sin(q_3)) - 0.0016*cos(q_1)*(1.0*cos(q_1)*cos(q_2)*cos(q_3) - 1.0*cos(q_1)*sin(q_2)*sin(q_3)))*(1.0*sin(q_1)*sin(q_2)*sin(q_3) - 1.0*cos(q_2)*cos(q_3)*sin(q_1)) - 1.0*(1.0*cos(q_1)*cos(q_2)*cos(q_3) - 1.0*cos(q_1)*sin(q_2)*sin(q_3))*(0.0016*cos(q_1)*(1.0*sin(q_1)*sin(q_2)*sin(q_3) - 1.0*cos(q_2)*cos(q_3)*sin(q_1)) + 0.0016*sin(q_1)*(cos(q_1)*cos(q_2)*cos(q_3) - 1.0*cos(q_1)*sin(q_2)*sin(q_3))) + 1.0*(0.0462*cos(q_1)*(1.0*cos(q_2)*sin(q_1)*sin(q_3) + 1.0*cos(q_3)*sin(q_1)*sin(q_2)) - 0.0462*sin(q_1)*(1.0*cos(q_1)*cos(q_2)*sin(q_3) + 1.0*cos(q_1)*cos(q_3)*sin(q_2)))*(1.0*cos(q_1)*cos(q_2)*sin(q_3) + 1.0*cos(q_1)*cos(q_3)*sin(q_2)) - 1.0*sin(q_1)*(0.0462*cos(q_1)^2 + 0.0462*sin(q_1)^2)) + 2.0*cos(q_1)*((0.0462*cos(q_2)*cos(q_3) - 0.0462*sin(q_2)*sin(q_3))*(1.0*sin(q_1)*sin(q_2)*sin(q_3) - 1.0*cos(q_2)*cos(q_3)*sin(q_1)) + (0.0462*cos(q_2)*sin(q_3) + 0.0462*cos(q_3)*sin(q_2))*(1.0*cos(q_2)*sin(q_1)*sin(q_3) + 1.0*cos(q_3)*sin(q_1)*sin(q_2)) - 1.0*(0.0016*cos(q_2)*cos(q_3) - 0.0016*sin(q_2)*sin(q_3))*(1.0*sin(q_1)*sin(q_2)*sin(q_3) - 1.0*cos(q_2)*cos(q_3)*sin(q_1)) - 1.0*(0.0016*cos(q_2)*sin(q_3) + 0.0016*cos(q_3)*sin(q_2))*(1.0*cos(q_2)*sin(q_1)*sin(q_3) + 1.0*cos(q_3)*sin(q_1)*sin(q_2))) - 1.0*sin(q_1)*((0.0016*cos(q_2)*cos(q_3) - 0.0016*sin(q_2)*sin(q_3))*(cos(q_1)*cos(q_2)*cos(q_3) - 1.0*cos(q_1)*sin(q_2)*sin(q_3)) - 1.0*(0.0016*cos(q_2)*sin(q_3) + 0.0016*cos(q_3)*sin(q_2))*(cos(q_1)*cos(q_2)*sin(q_3) + 1.0*cos(q_1)*cos(q_3)*sin(q_2)) - 1.0*(0.0462*cos(q_2)*cos(q_3) - 0.0462*sin(q_2)*sin(q_3))*(1.0*cos(q_1)*cos(q_2)*cos(q_3) - 1.0*cos(q_1)*sin(q_2)*sin(q_3)) + 1.0*(0.0462*cos(q_2)*sin(q_3) + 0.0462*cos(q_3)*sin(q_2))*(1.0*cos(q_1)*cos(q_2)*sin(q_3) + 1.0*cos(q_1)*cos(q_3)*sin(q_2))) - 1.0*sin(q_1)*((0.0016*cos(q_2)*cos(q_3) - 0.0016*sin(q_2)*sin(q_3))*(cos(q_1)*cos(q_2)*cos(q_3) - 1.0*cos(q_1)*sin(q_2)*sin(q_3)) - 1.0*(0.0016*cos(q_2)*sin(q_3) + 0.0016*cos(q_3)*sin(q_2))*(1.0*cos(q_1)*cos(q_2)*sin(q_3) + cos(q_1)*cos(q_3)*sin(q_2)) - 1.0*(0.0462*cos(q_2)*cos(q_3) - 0.0462*sin(q_2)*sin(q_3))*(1.0*cos(q_1)*cos(q_2)*cos(q_3) - 1.0*cos(q_1)*sin(q_2)*sin(q_3)) + 1.0*(0.0462*cos(q_2)*sin(q_3) + 0.0462*cos(q_3)*sin(q_2))*(1.0*cos(q_1)*cos(q_2)*sin(q_3) + 1.0*cos(q_1)*cos(q_3)*sin(q_2))) + 1.0*cos(q_1)*(1.0*sin(q_1)*(0.0462*cos(q_1)^2 + 0.0462*sin(q_1)^2) - 1.0*(0.0462*cos(q_1)*(1.0*cos(q_2)*sin(q_1)*sin(q_3) + 1.0*cos(q_3)*sin(q_1)*sin(q_2)) - 0.0462*sin(q_1)*(1.0*cos(q_1)*cos(q_2)*sin(q_3) + 1.0*cos(q_1)*cos(q_3)*sin(q_2)))*(1.0*cos(q_1)*cos(q_2)*sin(q_3) + 1.0*cos(q_1)*cos(q_3)*sin(q_2)) + (cos(q_1)*cos(q_2)*cos(q_3) - 1.0*cos(q_1)*sin(q_2)*sin(q_3))*(0.0016*cos(q_1)*(1.0*sin(q_1)*sin(q_2)*sin(q_3) - 1.0*cos(q_2)*cos(q_3)*sin(q_1)) + 0.0016*sin(q_1)*(cos(q_1)*cos(q_2)*cos(q_3) - 1.0*cos(q_1)*sin(q_2)*sin(q_3)))) + 2.0*cos(q_1)*(0.2723*cos(q_2)*cos(q_3) - 0.2723*sin(q_2)*sin(q_3))*(0.06029*cos(q_1) + 2.275*sin(q_1)*(0.2723*sin(q_2)*sin(q_3) - 1.0*cos(q_2)*(0.2723*cos(q_3) + 0.425))) + 2.0*sin(q_1)*(0.2723*cos(q_2)*cos(q_3) - 0.2723*sin(q_2)*sin(q_3))*(0.06029*sin(q_1) - 2.275*cos(q_1)*(0.2723*sin(q_2)*sin(q_3) - 1.0*cos(q_2)*(0.2723*cos(q_3) + 0.425)))),                                                                                                                                                                                                                                                                                                                                                                                                                                                                                                                                                                                                                                                                                                                                                                                                                                                                                                                                                                                                                                                                                                                                                                                                                                                                                                                                                                                                                                                                                                                                                                                                                                                                                                                                                                                                                                                                                                                                                                                                                                                                                                                                                                                                                                                                                                                                                                                                                                                                                                                                                                                                                                                                                                                              - 0.5*dq_1*(1.0*(1.0*cos(q_2)*cos(q_3) - 1.0*sin(q_2)*sin(q_3))*(0.0462*cos(q_2)*sin(q_3) + 0.0462*cos(q_3)*sin(q_2)) + 1.0*(1.0*cos(q_2)*sin(q_3) + 1.0*cos(q_3)*sin(q_2))*(0.0462*cos(q_2)*cos(q_3) - 0.0462*sin(q_2)*sin(q_3)) - 1.0*(1.0*cos(q_2)*cos(q_3) - 1.0*sin(q_2)*sin(q_3))*(0.0016*cos(q_2)*sin(q_3) + 0.0016*cos(q_3)*sin(q_2)) - 1.0*(1.0*cos(q_2)*sin(q_3) + 1.0*cos(q_3)*sin(q_2))*(0.0016*cos(q_2)*cos(q_3) - 0.0016*sin(q_2)*sin(q_3)) + 2.275*cos(q_1)*(0.0265*sin(q_1) - 1.0*cos(q_1)*(0.2723*sin(q_2)*sin(q_3) - 1.0*cos(q_2)*(0.2723*cos(q_3) + 0.425)))*(0.2723*cos(q_2)*sin(q_3) + 0.2723*cos(q_3)*sin(q_2)) - 2.275*sin(q_1)*(0.0265*cos(q_1) + 1.0*sin(q_1)*(0.2723*sin(q_2)*sin(q_3) - 1.0*cos(q_2)*(0.2723*cos(q_3) + 0.425)))*(0.2723*cos(q_2)*sin(q_3) + 0.2723*cos(q_3)*sin(q_2)) + 1.0*cos(q_1)*(0.2723*cos(q_2)*sin(q_3) + 0.2723*cos(q_3)*sin(q_2))*(0.06029*sin(q_1) - 2.275*cos(q_1)*(0.2723*sin(q_2)*sin(q_3) - 1.0*cos(q_2)*(0.2723*cos(q_3) + 0.425))) - 1.0*sin(q_1)*(0.2723*cos(q_2)*sin(q_3) + 0.2723*cos(q_3)*sin(q_2))*(0.06029*cos(q_1) + 2.275*sin(q_1)*(0.2723*sin(q_2)*sin(q_3) - 1.0*cos(q_2)*(0.2723*cos(q_3) + 0.425)))) - 0.5*dq_2*(1.0*sin(q_1)*((1.0*sin(q_1)*sin(q_2)*sin(q_3) - 1.0*cos(q_2)*cos(q_3)*sin(q_1))*(0.0016*cos(q_1)*(1.0*sin(q_1)*sin(q_2)*sin(q_3) - 1.0*cos(q_2)*cos(q_3)*sin(q_1)) + 0.0016*sin(q_1)*(cos(q_1)*cos(q_2)*cos(q_3) - 1.0*cos(q_1)*sin(q_2)*sin(q_3))) + 1.0*(0.0462*cos(q_1)*(1.0*cos(q_2)*sin(q_1)*sin(q_3) + 1.0*cos(q_3)*sin(q_1)*sin(q_2)) - 0.0462*sin(q_1)*(1.0*cos(q_1)*cos(q_2)*sin(q_3) + 1.0*cos(q_1)*cos(q_3)*sin(q_2)))*(1.0*cos(q_2)*sin(q_1)*sin(q_3) + 1.0*cos(q_3)*sin(q_1)*sin(q_2)) + 1.0*cos(q_1)*(0.0462*cos(q_1)^2 + 0.0462*sin(q_1)^2) + 1.0*(cos(q_1)*cos(q_2)*cos(q_3) - 1.0*cos(q_1)*sin(q_2)*sin(q_3))*(0.0016*cos(q_1)*(cos(q_1)*cos(q_2)*cos(q_3) - 1.0*cos(q_1)*sin(q_2)*sin(q_3)) - 0.0016*cos(q_1)*(1.0*cos(q_1)*cos(q_2)*cos(q_3) - 1.0*cos(q_1)*sin(q_2)*sin(q_3)))) - 1.0*sin(q_1)*((1.0*sin(q_1)*sin(q_2)*sin(q_3) - 1.0*cos(q_2)*cos(q_3)*sin(q_1))*(0.0016*cos(q_1)*(1.0*sin(q_1)*sin(q_2)*sin(q_3) - 1.0*cos(q_2)*cos(q_3)*sin(q_1)) + 0.0016*sin(q_1)*(cos(q_1)*cos(q_2)*cos(q_3) - 1.0*cos(q_1)*sin(q_2)*sin(q_3))) + (0.0462*cos(q_1)*(1.0*cos(q_2)*sin(q_1)*sin(q_3) + 1.0*cos(q_3)*sin(q_1)*sin(q_2)) - 0.0462*sin(q_1)*(1.0*cos(q_1)*cos(q_2)*sin(q_3) + 1.0*cos(q_1)*cos(q_3)*sin(q_2)))*(1.0*cos(q_2)*sin(q_1)*sin(q_3) + 1.0*cos(q_3)*sin(q_1)*sin(q_2)) + 1.0*cos(q_1)*(0.0462*cos(q_1)^2 + 0.0462*sin(q_1)^2)) + 1.0*cos(q_1)*((0.0016*cos(q_1)*(cos(q_1)*cos(q_2)*cos(q_3) - 1.0*cos(q_1)*sin(q_2)*sin(q_3)) - 0.0016*cos(q_1)*(1.0*cos(q_1)*cos(q_2)*cos(q_3) - 1.0*cos(q_1)*sin(q_2)*sin(q_3)))*(1.0*sin(q_1)*sin(q_2)*sin(q_3) - 1.0*cos(q_2)*cos(q_3)*sin(q_1)) - 1.0*(1.0*cos(q_1)*cos(q_2)*cos(q_3) - 1.0*cos(q_1)*sin(q_2)*sin(q_3))*(0.0016*cos(q_1)*(1.0*sin(q_1)*sin(q_2)*sin(q_3) - 1.0*cos(q_2)*cos(q_3)*sin(q_1)) + 0.0016*sin(q_1)*(cos(q_1)*cos(q_2)*cos(q_3) - 1.0*cos(q_1)*sin(q_2)*sin(q_3))) + 1.0*(0.0462*cos(q_1)*(1.0*cos(q_2)*sin(q_1)*sin(q_3) + 1.0*cos(q_3)*sin(q_1)*sin(q_2)) - 0.0462*sin(q_1)*(1.0*cos(q_1)*cos(q_2)*sin(q_3) + 1.0*cos(q_1)*cos(q_3)*sin(q_2)))*(1.0*cos(q_1)*cos(q_2)*sin(q_3) + 1.0*cos(q_1)*cos(q_3)*sin(q_2)) - 1.0*sin(q_1)*(0.0462*cos(q_1)^2 + 0.0462*sin(q_1)^2)) + 2.0*cos(q_1)*((0.0462*cos(q_2)*cos(q_3) - 0.0462*sin(q_2)*sin(q_3))*(1.0*sin(q_1)*sin(q_2)*sin(q_3) - 1.0*cos(q_2)*cos(q_3)*sin(q_1)) + (0.0462*cos(q_2)*sin(q_3) + 0.0462*cos(q_3)*sin(q_2))*(1.0*cos(q_2)*sin(q_1)*sin(q_3) + 1.0*cos(q_3)*sin(q_1)*sin(q_2)) - 1.0*(0.0016*cos(q_2)*cos(q_3) - 0.0016*sin(q_2)*sin(q_3))*(1.0*sin(q_1)*sin(q_2)*sin(q_3) - 1.0*cos(q_2)*cos(q_3)*sin(q_1)) - 1.0*(0.0016*cos(q_2)*sin(q_3) + 0.0016*cos(q_3)*sin(q_2))*(1.0*cos(q_2)*sin(q_1)*sin(q_3) + 1.0*cos(q_3)*sin(q_1)*sin(q_2))) - 1.0*sin(q_1)*((0.0016*cos(q_2)*cos(q_3) - 0.0016*sin(q_2)*sin(q_3))*(cos(q_1)*cos(q_2)*cos(q_3) - 1.0*cos(q_1)*sin(q_2)*sin(q_3)) - 1.0*(0.0016*cos(q_2)*sin(q_3) + 0.0016*cos(q_3)*sin(q_2))*(cos(q_1)*cos(q_2)*sin(q_3) + 1.0*cos(q_1)*cos(q_3)*sin(q_2)) - 1.0*(0.0462*cos(q_2)*cos(q_3) - 0.0462*sin(q_2)*sin(q_3))*(1.0*cos(q_1)*cos(q_2)*cos(q_3) - 1.0*cos(q_1)*sin(q_2)*sin(q_3)) + 1.0*(0.0462*cos(q_2)*sin(q_3) + 0.0462*cos(q_3)*sin(q_2))*(1.0*cos(q_1)*cos(q_2)*sin(q_3) + 1.0*cos(q_1)*cos(q_3)*sin(q_2))) - 1.0*sin(q_1)*((0.0016*cos(q_2)*cos(q_3) - 0.0016*sin(q_2)*sin(q_3))*(cos(q_1)*cos(q_2)*cos(q_3) - 1.0*cos(q_1)*sin(q_2)*sin(q_3)) - 1.0*(0.0016*cos(q_2)*sin(q_3) + 0.0016*cos(q_3)*sin(q_2))*(1.0*cos(q_1)*cos(q_2)*sin(q_3) + cos(q_1)*cos(q_3)*sin(q_2)) - 1.0*(0.0462*cos(q_2)*cos(q_3) - 0.0462*sin(q_2)*sin(q_3))*(1.0*cos(q_1)*cos(q_2)*cos(q_3) - 1.0*cos(q_1)*sin(q_2)*sin(q_3)) + 1.0*(0.0462*cos(q_2)*sin(q_3) + 0.0462*cos(q_3)*sin(q_2))*(1.0*cos(q_1)*cos(q_2)*sin(q_3) + 1.0*cos(q_1)*cos(q_3)*sin(q_2))) + 1.0*cos(q_1)*(1.0*sin(q_1)*(0.0462*cos(q_1)^2 + 0.0462*sin(q_1)^2) - 1.0*(0.0462*cos(q_1)*(1.0*cos(q_2)*sin(q_1)*sin(q_3) + 1.0*cos(q_3)*sin(q_1)*sin(q_2)) - 0.0462*sin(q_1)*(1.0*cos(q_1)*cos(q_2)*sin(q_3) + 1.0*cos(q_1)*cos(q_3)*sin(q_2)))*(1.0*cos(q_1)*cos(q_2)*sin(q_3) + 1.0*cos(q_1)*cos(q_3)*sin(q_2)) + (cos(q_1)*cos(q_2)*cos(q_3) - 1.0*cos(q_1)*sin(q_2)*sin(q_3))*(0.0016*cos(q_1)*(1.0*sin(q_1)*sin(q_2)*sin(q_3) - 1.0*cos(q_2)*cos(q_3)*sin(q_1)) + 0.0016*sin(q_1)*(cos(q_1)*cos(q_2)*cos(q_3) - 1.0*cos(q_1)*sin(q_2)*sin(q_3)))) + 2.0*cos(q_1)*(0.2723*cos(q_2)*cos(q_3) - 0.2723*sin(q_2)*sin(q_3))*(0.06029*cos(q_1) + 2.275*sin(q_1)*(0.2723*sin(q_2)*sin(q_3) - 1.0*cos(q_2)*(0.2723*cos(q_3) + 0.425))) + 2.0*sin(q_1)*(0.2723*cos(q_2)*cos(q_3) - 0.2723*sin(q_2)*sin(q_3))*(0.06029*sin(q_1) - 2.275*cos(q_1)*(0.2723*sin(q_2)*sin(q_3) - 1.0*cos(q_2)*(0.2723*cos(q_3) + 0.425)))) - 0.5*dq_3*(1.0*sin(q_1)*((1.0*sin(q_1)*sin(q_2)*sin(q_3) - 1.0*cos(q_2)*cos(q_3)*sin(q_1))*(0.0016*cos(q_1)*(1.0*sin(q_1)*sin(q_2)*sin(q_3) - 1.0*cos(q_2)*cos(q_3)*sin(q_1)) + 0.0016*sin(q_1)*(cos(q_1)*cos(q_2)*cos(q_3) - 1.0*cos(q_1)*sin(q_2)*sin(q_3))) + 1.0*(0.0462*cos(q_1)*(1.0*cos(q_2)*sin(q_1)*sin(q_3) + 1.0*cos(q_3)*sin(q_1)*sin(q_2)) - 0.0462*sin(q_1)*(1.0*cos(q_1)*cos(q_2)*sin(q_3) + 1.0*cos(q_1)*cos(q_3)*sin(q_2)))*(1.0*cos(q_2)*sin(q_1)*sin(q_3) + 1.0*cos(q_3)*sin(q_1)*sin(q_2)) + 1.0*cos(q_1)*(0.0462*cos(q_1)^2 + 0.0462*sin(q_1)^2) + 1.0*(cos(q_1)*cos(q_2)*cos(q_3) - 1.0*cos(q_1)*sin(q_2)*sin(q_3))*(0.0016*cos(q_1)*(cos(q_1)*cos(q_2)*cos(q_3) - 1.0*cos(q_1)*sin(q_2)*sin(q_3)) - 0.0016*cos(q_1)*(1.0*cos(q_1)*cos(q_2)*cos(q_3) - 1.0*cos(q_1)*sin(q_2)*sin(q_3)))) - 1.0*sin(q_1)*((1.0*sin(q_1)*sin(q_2)*sin(q_3) - 1.0*cos(q_2)*cos(q_3)*sin(q_1))*(0.0016*cos(q_1)*(1.0*sin(q_1)*sin(q_2)*sin(q_3) - 1.0*cos(q_2)*cos(q_3)*sin(q_1)) + 0.0016*sin(q_1)*(cos(q_1)*cos(q_2)*cos(q_3) - 1.0*cos(q_1)*sin(q_2)*sin(q_3))) + (0.0462*cos(q_1)*(1.0*cos(q_2)*sin(q_1)*sin(q_3) + 1.0*cos(q_3)*sin(q_1)*sin(q_2)) - 0.0462*sin(q_1)*(1.0*cos(q_1)*cos(q_2)*sin(q_3) + 1.0*cos(q_1)*cos(q_3)*sin(q_2)))*(1.0*cos(q_2)*sin(q_1)*sin(q_3) + 1.0*cos(q_3)*sin(q_1)*sin(q_2)) + 1.0*cos(q_1)*(0.0462*cos(q_1)^2 + 0.0462*sin(q_1)^2)) + 1.0*cos(q_1)*((0.0016*cos(q_1)*(cos(q_1)*cos(q_2)*cos(q_3) - 1.0*cos(q_1)*sin(q_2)*sin(q_3)) - 0.0016*cos(q_1)*(1.0*cos(q_1)*cos(q_2)*cos(q_3) - 1.0*cos(q_1)*sin(q_2)*sin(q_3)))*(1.0*sin(q_1)*sin(q_2)*sin(q_3) - 1.0*cos(q_2)*cos(q_3)*sin(q_1)) - 1.0*(1.0*cos(q_1)*cos(q_2)*cos(q_3) - 1.0*cos(q_1)*sin(q_2)*sin(q_3))*(0.0016*cos(q_1)*(1.0*sin(q_1)*sin(q_2)*sin(q_3) - 1.0*cos(q_2)*cos(q_3)*sin(q_1)) + 0.0016*sin(q_1)*(cos(q_1)*cos(q_2)*cos(q_3) - 1.0*cos(q_1)*sin(q_2)*sin(q_3))) + 1.0*(0.0462*cos(q_1)*(1.0*cos(q_2)*sin(q_1)*sin(q_3) + 1.0*cos(q_3)*sin(q_1)*sin(q_2)) - 0.0462*sin(q_1)*(1.0*cos(q_1)*cos(q_2)*sin(q_3) + 1.0*cos(q_1)*cos(q_3)*sin(q_2)))*(1.0*cos(q_1)*cos(q_2)*sin(q_3) + 1.0*cos(q_1)*cos(q_3)*sin(q_2)) - 1.0*sin(q_1)*(0.0462*cos(q_1)^2 + 0.0462*sin(q_1)^2)) + 2.0*cos(q_1)*((0.0462*cos(q_2)*cos(q_3) - 0.0462*sin(q_2)*sin(q_3))*(1.0*sin(q_1)*sin(q_2)*sin(q_3) - 1.0*cos(q_2)*cos(q_3)*sin(q_1)) + (0.0462*cos(q_2)*sin(q_3) + 0.0462*cos(q_3)*sin(q_2))*(1.0*cos(q_2)*sin(q_1)*sin(q_3) + 1.0*cos(q_3)*sin(q_1)*sin(q_2)) - 1.0*(0.0016*cos(q_2)*cos(q_3) - 0.0016*sin(q_2)*sin(q_3))*(1.0*sin(q_1)*sin(q_2)*sin(q_3) - 1.0*cos(q_2)*cos(q_3)*sin(q_1)) - 1.0*(0.0016*cos(q_2)*sin(q_3) + 0.0016*cos(q_3)*sin(q_2))*(1.0*cos(q_2)*sin(q_1)*sin(q_3) + 1.0*cos(q_3)*sin(q_1)*sin(q_2))) - 2.0*sin(q_1)*((0.0016*cos(q_2)*cos(q_3) - 0.0016*sin(q_2)*sin(q_3))*(cos(q_1)*cos(q_2)*cos(q_3) - 1.0*cos(q_1)*sin(q_2)*sin(q_3)) - 1.0*(0.0016*cos(q_2)*sin(q_3) + 0.0016*cos(q_3)*sin(q_2))*(cos(q_1)*cos(q_2)*sin(q_3) + 1.0*cos(q_1)*cos(q_3)*sin(q_2)) - 1.0*(0.0462*cos(q_2)*cos(q_3) - 0.0462*sin(q_2)*sin(q_3))*(1.0*cos(q_1)*cos(q_2)*cos(q_3) - 1.0*cos(q_1)*sin(q_2)*sin(q_3)) + 1.0*(0.0462*cos(q_2)*sin(q_3) + 0.0462*cos(q_3)*sin(q_2))*(1.0*cos(q_1)*cos(q_2)*sin(q_3) + 1.0*cos(q_1)*cos(q_3)*sin(q_2))) + 1.0*cos(q_1)*(1.0*sin(q_1)*(0.0462*cos(q_1)^2 + 0.0462*sin(q_1)^2) - 1.0*(0.0462*cos(q_1)*(1.0*cos(q_2)*sin(q_1)*sin(q_3) + 1.0*cos(q_3)*sin(q_1)*sin(q_2)) - 0.0462*sin(q_1)*(1.0*cos(q_1)*cos(q_2)*sin(q_3) + 1.0*cos(q_1)*cos(q_3)*sin(q_2)))*(1.0*cos(q_1)*cos(q_2)*sin(q_3) + 1.0*cos(q_1)*cos(q_3)*sin(q_2)) + (cos(q_1)*cos(q_2)*cos(q_3) - 1.0*cos(q_1)*sin(q_2)*sin(q_3))*(0.0016*cos(q_1)*(1.0*sin(q_1)*sin(q_2)*sin(q_3) - 1.0*cos(q_2)*cos(q_3)*sin(q_1)) + 0.0016*sin(q_1)*(cos(q_1)*cos(q_2)*cos(q_3) - 1.0*cos(q_1)*sin(q_2)*sin(q_3)))) + 2.0*cos(q_1)*(0.2723*cos(q_2)*cos(q_3) - 0.2723*sin(q_2)*sin(q_3))*(0.06029*cos(q_1) + 2.275*sin(q_1)*(0.2723*sin(q_2)*sin(q_3) - 1.0*cos(q_2)*(0.2723*cos(q_3) + 0.425))) + 2.0*sin(q_1)*(0.2723*cos(q_2)*cos(q_3) - 0.2723*sin(q_2)*sin(q_3))*(0.06029*sin(q_1) - 2.275*cos(q_1)*(0.2723*sin(q_2)*sin(q_3) - 1.0*cos(q_2)*(0.2723*cos(q_3) + 0.425))))
0.5*dq_2*(1.0*sin(q_1)*((1.0*sin(q_1)*sin(q_2)*sin(q_3) - 1.0*cos(q_2)*cos(q_3)*sin(q_1))*(0.0016*cos(q_1)*(1.0*sin(q_1)*sin(q_2)*sin(q_3) - 1.0*cos(q_2)*cos(q_3)*sin(q_1)) + 0.0016*sin(q_1)*(cos(q_1)*cos(q_2)*cos(q_3) - 1.0*cos(q_1)*sin(q_2)*sin(q_3))) + 1.0*(0.0462*cos(q_1)*(1.0*cos(q_2)*sin(q_1)*sin(q_3) + 1.0*cos(q_3)*sin(q_1)*sin(q_2)) - 0.0462*sin(q_1)*(1.0*cos(q_1)*cos(q_2)*sin(q_3) + 1.0*cos(q_1)*cos(q_3)*sin(q_2)))*(1.0*cos(q_2)*sin(q_1)*sin(q_3) + 1.0*cos(q_3)*sin(q_1)*sin(q_2)) + 1.0*cos(q_1)*(0.0462*cos(q_1)^2 + 0.0462*sin(q_1)^2) + 1.0*(cos(q_1)*cos(q_2)*cos(q_3) - 1.0*cos(q_1)*sin(q_2)*sin(q_3))*(0.0016*cos(q_1)*(cos(q_1)*cos(q_2)*cos(q_3) - 1.0*cos(q_1)*sin(q_2)*sin(q_3)) - 0.0016*cos(q_1)*(1.0*cos(q_1)*cos(q_2)*cos(q_3) - 1.0*cos(q_1)*sin(q_2)*sin(q_3)))) - 1.0*sin(q_1)*((1.0*sin(q_1)*sin(q_2)*sin(q_3) - 1.0*cos(q_2)*cos(q_3)*sin(q_1))*(0.0016*cos(q_1)*(1.0*sin(q_1)*sin(q_2)*sin(q_3) - 1.0*cos(q_2)*cos(q_3)*sin(q_1)) + 0.0016*sin(q_1)*(cos(q_1)*cos(q_2)*cos(q_3) - 1.0*cos(q_1)*sin(q_2)*sin(q_3))) + (0.0462*cos(q_1)*(1.0*cos(q_2)*sin(q_1)*sin(q_3) + 1.0*cos(q_3)*sin(q_1)*sin(q_2)) - 0.0462*sin(q_1)*(1.0*cos(q_1)*cos(q_2)*sin(q_3) + 1.0*cos(q_1)*cos(q_3)*sin(q_2)))*(1.0*cos(q_2)*sin(q_1)*sin(q_3) + 1.0*cos(q_3)*sin(q_1)*sin(q_2)) + 1.0*cos(q_1)*(0.0462*cos(q_1)^2 + 0.0462*sin(q_1)^2)) + 1.0*cos(q_1)*((0.0016*cos(q_1)*(cos(q_1)*cos(q_2)*cos(q_3) - 1.0*cos(q_1)*sin(q_2)*sin(q_3)) - 0.0016*cos(q_1)*(1.0*cos(q_1)*cos(q_2)*cos(q_3) - 1.0*cos(q_1)*sin(q_2)*sin(q_3)))*(1.0*sin(q_1)*sin(q_2)*sin(q_3) - 1.0*cos(q_2)*cos(q_3)*sin(q_1)) - 1.0*(1.0*cos(q_1)*cos(q_2)*cos(q_3) - 1.0*cos(q_1)*sin(q_2)*sin(q_3))*(0.0016*cos(q_1)*(1.0*sin(q_1)*sin(q_2)*sin(q_3) - 1.0*cos(q_2)*cos(q_3)*sin(q_1)) + 0.0016*sin(q_1)*(cos(q_1)*cos(q_2)*cos(q_3) - 1.0*cos(q_1)*sin(q_2)*sin(q_3))) + 1.0*(0.0462*cos(q_1)*(1.0*cos(q_2)*sin(q_1)*sin(q_3) + 1.0*cos(q_3)*sin(q_1)*sin(q_2)) - 0.0462*sin(q_1)*(1.0*cos(q_1)*cos(q_2)*sin(q_3) + 1.0*cos(q_1)*cos(q_3)*sin(q_2)))*(1.0*cos(q_1)*cos(q_2)*sin(q_3) + 1.0*cos(q_1)*cos(q_3)*sin(q_2)) - 1.0*sin(q_1)*(0.0462*cos(q_1)^2 + 0.0462*sin(q_1)^2)) + 1.0*cos(q_1)*(1.0*sin(q_1)*(0.0462*cos(q_1)^2 + 0.0462*sin(q_1)^2) - 1.0*(0.0462*cos(q_1)*(1.0*cos(q_2)*sin(q_1)*sin(q_3) + 1.0*cos(q_3)*sin(q_1)*sin(q_2)) - 0.0462*sin(q_1)*(1.0*cos(q_1)*cos(q_2)*sin(q_3) + 1.0*cos(q_1)*cos(q_3)*sin(q_2)))*(1.0*cos(q_1)*cos(q_2)*sin(q_3) + 1.0*cos(q_1)*cos(q_3)*sin(q_2)) + (cos(q_1)*cos(q_2)*cos(q_3) - 1.0*cos(q_1)*sin(q_2)*sin(q_3))*(0.0016*cos(q_1)*(1.0*sin(q_1)*sin(q_2)*sin(q_3) - 1.0*cos(q_2)*cos(q_3)*sin(q_1)) + 0.0016*sin(q_1)*(cos(q_1)*cos(q_2)*cos(q_3) - 1.0*cos(q_1)*sin(q_2)*sin(q_3))))) - 0.5*dq_1*(0.0114*cos(q_2)*sin(q_2) - 2.0*(1.0*cos(q_2)*sin(q_3) + 1.0*cos(q_3)*sin(q_2))*(0.0016*cos(q_1)*(cos(q_1)*cos(q_2)*cos(q_3) - 1.0*cos(q_1)*sin(q_2)*sin(q_3)) - 0.0016*cos(q_1)*(1.0*cos(q_1)*cos(q_2)*cos(q_3) - 1.0*cos(q_1)*sin(q_2)*sin(q_3))) - 1.0*(1.0*cos(q_2)*cos(q_3) - 1.0*sin(q_2)*sin(q_3))*(0.0462*cos(q_2)*sin(q_3) + 0.0462*cos(q_3)*sin(q_2)) - 1.0*(1.0*cos(q_2)*sin(q_3) + 1.0*cos(q_3)*sin(q_2))*(0.0462*cos(q_2)*cos(q_3) - 0.0462*sin(q_2)*sin(q_3)) + 1.0*(1.0*cos(q_2)*cos(q_3) - 1.0*sin(q_2)*sin(q_3))*(0.0016*cos(q_2)*sin(q_3) + 0.0016*cos(q_3)*sin(q_2)) + 1.0*(1.0*cos(q_2)*sin(q_3) + 1.0*cos(q_3)*sin(q_2))*(0.0016*cos(q_2)*cos(q_3) - 0.0016*sin(q_2)*sin(q_3)) - 1.784*cos(q_1)*sin(q_2)*(0.1134*sin(q_1) + 0.2125*cos(q_1)*cos(q_2)) - 0.2125*cos(q_1)*sin(q_2)*(0.9514*sin(q_1) + 1.784*cos(q_1)*cos(q_2)) + 1.784*sin(q_1)*sin(q_2)*(0.1134*cos(q_1) - 0.2125*cos(q_2)*sin(q_1)) + 0.2125*sin(q_1)*sin(q_2)*(0.9514*cos(q_1) - 1.784*cos(q_2)*sin(q_1)) - 2.275*cos(q_1)*(0.0265*sin(q_1) - 1.0*cos(q_1)*(0.2723*sin(q_2)*sin(q_3) - 1.0*cos(q_2)*(0.2723*cos(q_3) + 0.425)))*(0.2723*cos(q_2)*sin(q_3) + 1.0*sin(q_2)*(0.2723*cos(q_3) + 0.425)) + 2.275*sin(q_1)*(0.0265*cos(q_1) + 1.0*sin(q_1)*(0.2723*sin(q_2)*sin(q_3) - 1.0*cos(q_2)*(0.2723*cos(q_3) + 0.425)))*(0.2723*cos(q_2)*sin(q_3) + 1.0*sin(q_2)*(0.2723*cos(q_3) + 0.425)) - 1.0*cos(q_1)*(0.06029*sin(q_1) - 2.275*cos(q_1)*(0.2723*sin(q_2)*sin(q_3) - 1.0*cos(q_2)*(0.2723*cos(q_3) + 0.425)))*(0.2723*cos(q_2)*sin(q_3) + 1.0*sin(q_2)*(0.2723*cos(q_3) + 0.425)) + 1.0*sin(q_1)*(0.06029*cos(q_1) + 2.275*sin(q_1)*(0.2723*sin(q_2)*sin(q_3) - 1.0*cos(q_2)*(0.2723*cos(q_3) + 0.425)))*(0.2723*cos(q_2)*sin(q_3) + 1.0*sin(q_2)*(0.2723*cos(q_3) + 0.425))) + 0.5*dq_3*(1.0*sin(q_1)*((1.0*sin(q_1)*sin(q_2)*sin(q_3) - 1.0*cos(q_2)*cos(q_3)*sin(q_1))*(0.0016*cos(q_1)*(1.0*sin(q_1)*sin(q_2)*sin(q_3) - 1.0*cos(q_2)*cos(q_3)*sin(q_1)) + 0.0016*sin(q_1)*(cos(q_1)*cos(q_2)*cos(q_3) - 1.0*cos(q_1)*sin(q_2)*sin(q_3))) + 1.0*(0.0462*cos(q_1)*(1.0*cos(q_2)*sin(q_1)*sin(q_3) + 1.0*cos(q_3)*sin(q_1)*sin(q_2)) - 0.0462*sin(q_1)*(1.0*cos(q_1)*cos(q_2)*sin(q_3) + 1.0*cos(q_1)*cos(q_3)*sin(q_2)))*(1.0*cos(q_2)*sin(q_1)*sin(q_3) + 1.0*cos(q_3)*sin(q_1)*sin(q_2)) + 1.0*cos(q_1)*(0.0462*cos(q_1)^2 + 0.0462*sin(q_1)^2) + 1.0*(cos(q_1)*cos(q_2)*cos(q_3) - 1.0*cos(q_1)*sin(q_2)*sin(q_3))*(0.0016*cos(q_1)*(cos(q_1)*cos(q_2)*cos(q_3) - 1.0*cos(q_1)*sin(q_2)*sin(q_3)) - 0.0016*cos(q_1)*(1.0*cos(q_1)*cos(q_2)*cos(q_3) - 1.0*cos(q_1)*sin(q_2)*sin(q_3)))) - 1.0*sin(q_1)*((1.0*sin(q_1)*sin(q_2)*sin(q_3) - 1.0*cos(q_2)*cos(q_3)*sin(q_1))*(0.0016*cos(q_1)*(1.0*sin(q_1)*sin(q_2)*sin(q_3) - 1.0*cos(q_2)*cos(q_3)*sin(q_1)) + 0.0016*sin(q_1)*(cos(q_1)*cos(q_2)*cos(q_3) - 1.0*cos(q_1)*sin(q_2)*sin(q_3))) + (0.0462*cos(q_1)*(1.0*cos(q_2)*sin(q_1)*sin(q_3) + 1.0*cos(q_3)*sin(q_1)*sin(q_2)) - 0.0462*sin(q_1)*(1.0*cos(q_1)*cos(q_2)*sin(q_3) + 1.0*cos(q_1)*cos(q_3)*sin(q_2)))*(1.0*cos(q_2)*sin(q_1)*sin(q_3) + 1.0*cos(q_3)*sin(q_1)*sin(q_2)) + 1.0*cos(q_1)*(0.0462*cos(q_1)^2 + 0.0462*sin(q_1)^2)) + 1.0*cos(q_1)*((0.0016*cos(q_1)*(cos(q_1)*cos(q_2)*cos(q_3) - 1.0*cos(q_1)*sin(q_2)*sin(q_3)) - 0.0016*cos(q_1)*(1.0*cos(q_1)*cos(q_2)*cos(q_3) - 1.0*cos(q_1)*sin(q_2)*sin(q_3)))*(1.0*sin(q_1)*sin(q_2)*sin(q_3) - 1.0*cos(q_2)*cos(q_3)*sin(q_1)) - 1.0*(1.0*cos(q_1)*cos(q_2)*cos(q_3) - 1.0*cos(q_1)*sin(q_2)*sin(q_3))*(0.0016*cos(q_1)*(1.0*sin(q_1)*sin(q_2)*sin(q_3) - 1.0*cos(q_2)*cos(q_3)*sin(q_1)) + 0.0016*sin(q_1)*(cos(q_1)*cos(q_2)*cos(q_3) - 1.0*cos(q_1)*sin(q_2)*sin(q_3))) + 1.0*(0.0462*cos(q_1)*(1.0*cos(q_2)*sin(q_1)*sin(q_3) + 1.0*cos(q_3)*sin(q_1)*sin(q_2)) - 0.0462*sin(q_1)*(1.0*cos(q_1)*cos(q_2)*sin(q_3) + 1.0*cos(q_1)*cos(q_3)*sin(q_2)))*(1.0*cos(q_1)*cos(q_2)*sin(q_3) + 1.0*cos(q_1)*cos(q_3)*sin(q_2)) - 1.0*sin(q_1)*(0.0462*cos(q_1)^2 + 0.0462*sin(q_1)^2)) + 1.0*(1.0*cos(q_2)*sin(q_3) + 1.0*cos(q_3)*sin(q_2))*(0.0016*cos(q_1)*(1.0*cos(q_2)*sin(q_1)*sin(q_3) + 1.0*cos(q_3)*sin(q_1)*sin(q_2)) - 0.0016*sin(q_1)*(cos(q_1)*cos(q_2)*sin(q_3) + 1.0*cos(q_1)*cos(q_3)*sin(q_2))) - 1.0*(1.0*cos(q_2)*sin(q_3) + 1.0*cos(q_3)*sin(q_2))*(0.0016*cos(q_1)*(1.0*cos(q_2)*sin(q_1)*sin(q_3) + 1.0*cos(q_3)*sin(q_1)*sin(q_2)) - 0.0016*sin(q_1)*(1.0*cos(q_1)*cos(q_2)*sin(q_3) + cos(q_1)*cos(q_3)*sin(q_2))) + 1.0*cos(q_1)*(1.0*sin(q_1)*(0.0462*cos(q_1)^2 + 0.0462*sin(q_1)^2) - 1.0*(0.0462*cos(q_1)*(1.0*cos(q_2)*sin(q_1)*sin(q_3) + 1.0*cos(q_3)*sin(q_1)*sin(q_2)) - 0.0462*sin(q_1)*(1.0*cos(q_1)*cos(q_2)*sin(q_3) + 1.0*cos(q_1)*cos(q_3)*sin(q_2)))*(1.0*cos(q_1)*cos(q_2)*sin(q_3) + 1.0*cos(q_1)*cos(q_3)*sin(q_2)) + (cos(q_1)*cos(q_2)*cos(q_3) - 1.0*cos(q_1)*sin(q_2)*sin(q_3))*(0.0016*cos(q_1)*(1.0*sin(q_1)*sin(q_2)*sin(q_3) - 1.0*cos(q_2)*cos(q_3)*sin(q_1)) + 0.0016*sin(q_1)*(cos(q_1)*cos(q_2)*cos(q_3) - 1.0*cos(q_1)*sin(q_2)*sin(q_3))))),                                                                                                                                                                                                                                                                                                                                                                                                                                                                                                                                                                                                                                                                                                                                                                                                                                                                                                                                                                                                                                                                                                                                                                                                                                                                                 0.5*dq_1*(1.0*sin(q_1)*((1.0*sin(q_1)*sin(q_2)*sin(q_3) - 1.0*cos(q_2)*cos(q_3)*sin(q_1))*(0.0016*cos(q_1)*(1.0*sin(q_1)*sin(q_2)*sin(q_3) - 1.0*cos(q_2)*cos(q_3)*sin(q_1)) + 0.0016*sin(q_1)*(cos(q_1)*cos(q_2)*cos(q_3) - 1.0*cos(q_1)*sin(q_2)*sin(q_3))) + 1.0*(0.0462*cos(q_1)*(1.0*cos(q_2)*sin(q_1)*sin(q_3) + 1.0*cos(q_3)*sin(q_1)*sin(q_2)) - 0.0462*sin(q_1)*(1.0*cos(q_1)*cos(q_2)*sin(q_3) + 1.0*cos(q_1)*cos(q_3)*sin(q_2)))*(1.0*cos(q_2)*sin(q_1)*sin(q_3) + 1.0*cos(q_3)*sin(q_1)*sin(q_2)) + 1.0*cos(q_1)*(0.0462*cos(q_1)^2 + 0.0462*sin(q_1)^2) + 1.0*(cos(q_1)*cos(q_2)*cos(q_3) - 1.0*cos(q_1)*sin(q_2)*sin(q_3))*(0.0016*cos(q_1)*(cos(q_1)*cos(q_2)*cos(q_3) - 1.0*cos(q_1)*sin(q_2)*sin(q_3)) - 0.0016*cos(q_1)*(1.0*cos(q_1)*cos(q_2)*cos(q_3) - 1.0*cos(q_1)*sin(q_2)*sin(q_3)))) - 1.0*sin(q_1)*((1.0*sin(q_1)*sin(q_2)*sin(q_3) - 1.0*cos(q_2)*cos(q_3)*sin(q_1))*(0.0016*cos(q_1)*(1.0*sin(q_1)*sin(q_2)*sin(q_3) - 1.0*cos(q_2)*cos(q_3)*sin(q_1)) + 0.0016*sin(q_1)*(cos(q_1)*cos(q_2)*cos(q_3) - 1.0*cos(q_1)*sin(q_2)*sin(q_3))) + (0.0462*cos(q_1)*(1.0*cos(q_2)*sin(q_1)*sin(q_3) + 1.0*cos(q_3)*sin(q_1)*sin(q_2)) - 0.0462*sin(q_1)*(1.0*cos(q_1)*cos(q_2)*sin(q_3) + 1.0*cos(q_1)*cos(q_3)*sin(q_2)))*(1.0*cos(q_2)*sin(q_1)*sin(q_3) + 1.0*cos(q_3)*sin(q_1)*sin(q_2)) + 1.0*cos(q_1)*(0.0462*cos(q_1)^2 + 0.0462*sin(q_1)^2)) + 1.0*cos(q_1)*((0.0016*cos(q_1)*(cos(q_1)*cos(q_2)*cos(q_3) - 1.0*cos(q_1)*sin(q_2)*sin(q_3)) - 0.0016*cos(q_1)*(1.0*cos(q_1)*cos(q_2)*cos(q_3) - 1.0*cos(q_1)*sin(q_2)*sin(q_3)))*(1.0*sin(q_1)*sin(q_2)*sin(q_3) - 1.0*cos(q_2)*cos(q_3)*sin(q_1)) - 1.0*(1.0*cos(q_1)*cos(q_2)*cos(q_3) - 1.0*cos(q_1)*sin(q_2)*sin(q_3))*(0.0016*cos(q_1)*(1.0*sin(q_1)*sin(q_2)*sin(q_3) - 1.0*cos(q_2)*cos(q_3)*sin(q_1)) + 0.0016*sin(q_1)*(cos(q_1)*cos(q_2)*cos(q_3) - 1.0*cos(q_1)*sin(q_2)*sin(q_3))) + 1.0*(0.0462*cos(q_1)*(1.0*cos(q_2)*sin(q_1)*sin(q_3) + 1.0*cos(q_3)*sin(q_1)*sin(q_2)) - 0.0462*sin(q_1)*(1.0*cos(q_1)*cos(q_2)*sin(q_3) + 1.0*cos(q_1)*cos(q_3)*sin(q_2)))*(1.0*cos(q_1)*cos(q_2)*sin(q_3) + 1.0*cos(q_1)*cos(q_3)*sin(q_2)) - 1.0*sin(q_1)*(0.0462*cos(q_1)^2 + 0.0462*sin(q_1)^2)) + 1.0*cos(q_1)*((0.0462*cos(q_2)*cos(q_3) - 0.0462*sin(q_2)*sin(q_3))*(1.0*sin(q_1)*sin(q_2)*sin(q_3) - 1.0*cos(q_2)*cos(q_3)*sin(q_1)) + (0.0462*cos(q_2)*sin(q_3) + 0.0462*cos(q_3)*sin(q_2))*(1.0*cos(q_2)*sin(q_1)*sin(q_3) + 1.0*cos(q_3)*sin(q_1)*sin(q_2)) - 1.0*(0.0016*cos(q_2)*cos(q_3) - 0.0016*sin(q_2)*sin(q_3))*(1.0*sin(q_1)*sin(q_2)*sin(q_3) - 1.0*cos(q_2)*cos(q_3)*sin(q_1)) - 1.0*(0.0016*cos(q_2)*sin(q_3) + 0.0016*cos(q_3)*sin(q_2))*(1.0*cos(q_2)*sin(q_1)*sin(q_3) + 1.0*cos(q_3)*sin(q_1)*sin(q_2))) + 1.0*(1.0*cos(q_2)*cos(q_3) - 1.0*sin(q_2)*sin(q_3))*(0.0016*cos(q_1)*(1.0*sin(q_1)*sin(q_2)*sin(q_3) - 1.0*cos(q_2)*cos(q_3)*sin(q_1)) + 0.0016*sin(q_1)*(cos(q_1)*cos(q_2)*cos(q_3) - 1.0*cos(q_1)*sin(q_2)*sin(q_3))) + 1.0*(1.0*cos(q_2)*sin(q_3) + 1.0*cos(q_3)*sin(q_2))*(0.0016*cos(q_1)*(1.0*cos(q_2)*sin(q_1)*sin(q_3) + 1.0*cos(q_3)*sin(q_1)*sin(q_2)) - 0.0016*sin(q_1)*(1.0*cos(q_1)*cos(q_2)*sin(q_3) + cos(q_1)*cos(q_3)*sin(q_2))) - 1.0*(1.0*cos(q_2)*cos(q_3) - 1.0*sin(q_2)*sin(q_3))*(0.0462*cos(q_1)*(1.0*sin(q_1)*sin(q_2)*sin(q_3) - 1.0*cos(q_2)*cos(q_3)*sin(q_1)) + 0.0462*sin(q_1)*(1.0*cos(q_1)*cos(q_2)*cos(q_3) - 1.0*cos(q_1)*sin(q_2)*sin(q_3))) - 1.0*(1.0*cos(q_2)*sin(q_3) + 1.0*cos(q_3)*sin(q_2))*(0.0462*cos(q_1)*(1.0*cos(q_2)*sin(q_1)*sin(q_3) + 1.0*cos(q_3)*sin(q_1)*sin(q_2)) - 0.0462*sin(q_1)*(1.0*cos(q_1)*cos(q_2)*sin(q_3) + 1.0*cos(q_1)*cos(q_3)*sin(q_2))) - 1.0*sin(q_1)*((0.0016*cos(q_2)*cos(q_3) - 0.0016*sin(q_2)*sin(q_3))*(cos(q_1)*cos(q_2)*cos(q_3) - 1.0*cos(q_1)*sin(q_2)*sin(q_3)) - 1.0*(0.0016*cos(q_2)*sin(q_3) + 0.0016*cos(q_3)*sin(q_2))*(1.0*cos(q_1)*cos(q_2)*sin(q_3) + cos(q_1)*cos(q_3)*sin(q_2)) - 1.0*(0.0462*cos(q_2)*cos(q_3) - 0.0462*sin(q_2)*sin(q_3))*(1.0*cos(q_1)*cos(q_2)*cos(q_3) - 1.0*cos(q_1)*sin(q_2)*sin(q_3)) + 1.0*(0.0462*cos(q_2)*sin(q_3) + 0.0462*cos(q_3)*sin(q_2))*(1.0*cos(q_1)*cos(q_2)*sin(q_3) + 1.0*cos(q_1)*cos(q_3)*sin(q_2))) + 1.0*cos(q_1)*(1.0*sin(q_1)*(0.0462*cos(q_1)^2 + 0.0462*sin(q_1)^2) - 1.0*(0.0462*cos(q_1)*(1.0*cos(q_2)*sin(q_1)*sin(q_3) + 1.0*cos(q_3)*sin(q_1)*sin(q_2)) - 0.0462*sin(q_1)*(1.0*cos(q_1)*cos(q_2)*sin(q_3) + 1.0*cos(q_1)*cos(q_3)*sin(q_2)))*(1.0*cos(q_1)*cos(q_2)*sin(q_3) + 1.0*cos(q_1)*cos(q_3)*sin(q_2)) + (cos(q_1)*cos(q_2)*cos(q_3) - 1.0*cos(q_1)*sin(q_2)*sin(q_3))*(0.0016*cos(q_1)*(1.0*sin(q_1)*sin(q_2)*sin(q_3) - 1.0*cos(q_2)*cos(q_3)*sin(q_1)) + 0.0016*sin(q_1)*(cos(q_1)*cos(q_2)*cos(q_3) - 1.0*cos(q_1)*sin(q_2)*sin(q_3)))) - 1.784*cos(q_1)*cos(q_2)*(0.1134*cos(q_1) - 0.2125*cos(q_2)*sin(q_1)) + 0.2125*cos(q_1)*cos(q_2)*(0.9514*cos(q_1) - 1.784*cos(q_2)*sin(q_1)) - 1.784*cos(q_2)*sin(q_1)*(0.1134*sin(q_1) + 0.2125*cos(q_1)*cos(q_2)) + 0.2125*cos(q_2)*sin(q_1)*(0.9514*sin(q_1) + 1.784*cos(q_1)*cos(q_2)) + 2.275*cos(q_1)*(0.0265*cos(q_1) + 1.0*sin(q_1)*(0.2723*sin(q_2)*sin(q_3) - 1.0*cos(q_2)*(0.2723*cos(q_3) + 0.425)))*(0.2723*sin(q_2)*sin(q_3) - 1.0*cos(q_2)*(0.2723*cos(q_3) + 0.425)) + 2.275*sin(q_1)*(0.0265*sin(q_1) - 1.0*cos(q_1)*(0.2723*sin(q_2)*sin(q_3) - 1.0*cos(q_2)*(0.2723*cos(q_3) + 0.425)))*(0.2723*sin(q_2)*sin(q_3) - 1.0*cos(q_2)*(0.2723*cos(q_3) + 0.425)) - 1.0*cos(q_1)*(0.06029*cos(q_1) + 2.275*sin(q_1)*(0.2723*sin(q_2)*sin(q_3) - 1.0*cos(q_2)*(0.2723*cos(q_3) + 0.425)))*(0.2723*sin(q_2)*sin(q_3) - 1.0*cos(q_2)*(0.2723*cos(q_3) + 0.425)) - 1.0*sin(q_1)*(0.06029*sin(q_1) - 2.275*cos(q_1)*(0.2723*sin(q_2)*sin(q_3) - 1.0*cos(q_2)*(0.2723*cos(q_3) + 0.425)))*(0.2723*sin(q_2)*sin(q_3) - 1.0*cos(q_2)*(0.2723*cos(q_3) + 0.425))) + 0.5*dq_3*(2.0*(0.2723*cos(q_2)*sin(q_3) + 0.2723*cos(q_3)*sin(q_2))*(0.6195*sin(q_2)*sin(q_3) - 2.275*cos(q_2)*(0.2723*cos(q_3) + 0.425)) - 1.0*(0.2723*cos(q_2)*cos(q_3) - 0.2723*sin(q_2)*sin(q_3))*(0.6195*cos(q_2)*sin(q_3) + 2.275*sin(q_2)*(0.2723*cos(q_3) + 0.425)) + 1.0*(0.6195*cos(q_2)*cos(q_3) - 0.6195*sin(q_2)*sin(q_3))*(0.2723*cos(q_2)*sin(q_3) + 1.0*sin(q_2)*(0.2723*cos(q_3) + 0.425)) - 1.0*(0.6195*cos(q_2)*sin(q_3) + 0.6195*cos(q_3)*sin(q_2))*(0.2723*sin(q_2)*sin(q_3) - 1.0*cos(q_2)*(0.2723*cos(q_3) + 0.425)) + (0.6195*cos(q_2)*sin(q_3) + 0.6195*cos(q_3)*sin(q_2))*(0.2723*sin(q_2)*sin(q_3) - 1.0*cos(q_2)*(0.2723*cos(q_3) + 0.425)) + 1.0*cos(q_1)*((1.0*cos(q_2)*sin(q_1)*sin(q_3) + 1.0*cos(q_3)*sin(q_1)*sin(q_2))*(0.0016*cos(q_1)*(1.0*sin(q_1)*sin(q_2)*sin(q_3) - 1.0*cos(q_2)*cos(q_3)*sin(q_1)) + 0.0016*sin(q_1)*(cos(q_1)*cos(q_2)*cos(q_3) - 1.0*cos(q_1)*sin(q_2)*sin(q_3))) + (1.0*sin(q_1)*sin(q_2)*sin(q_3) - 1.0*cos(q_2)*cos(q_3)*sin(q_1))*(0.0016*cos(q_1)*(1.0*cos(q_2)*sin(q_1)*sin(q_3) + 1.0*cos(q_3)*sin(q_1)*sin(q_2)) - 0.0016*sin(q_1)*(cos(q_1)*cos(q_2)*sin(q_3) + 1.0*cos(q_1)*cos(q_3)*sin(q_2))) - 1.0*(0.0462*cos(q_1)*(1.0*cos(q_2)*sin(q_1)*sin(q_3) + 1.0*cos(q_3)*sin(q_1)*sin(q_2)) - 0.0462*sin(q_1)*(1.0*cos(q_1)*cos(q_2)*sin(q_3) + 1.0*cos(q_1)*cos(q_3)*sin(q_2)))*(1.0*sin(q_1)*sin(q_2)*sin(q_3) - 1.0*cos(q_2)*cos(q_3)*sin(q_1)) - 1.0*(0.0462*cos(q_1)*(1.0*sin(q_1)*sin(q_2)*sin(q_3) - 1.0*cos(q_2)*cos(q_3)*sin(q_1)) + 0.0462*sin(q_1)*(1.0*cos(q_1)*cos(q_2)*cos(q_3) - 1.0*cos(q_1)*sin(q_2)*sin(q_3)))*(1.0*cos(q_2)*sin(q_1)*sin(q_3) + 1.0*cos(q_3)*sin(q_1)*sin(q_2))) - 1.0*sin(q_1)*(1.0*(0.0462*cos(q_1)*(1.0*cos(q_2)*sin(q_1)*sin(q_3) + 1.0*cos(q_3)*sin(q_1)*sin(q_2)) - 0.0462*sin(q_1)*(1.0*cos(q_1)*cos(q_2)*sin(q_3) + 1.0*cos(q_1)*cos(q_3)*sin(q_2)))*(1.0*cos(q_1)*cos(q_2)*cos(q_3) - 1.0*cos(q_1)*sin(q_2)*sin(q_3)) - 1.0*(0.0462*cos(q_1)*(1.0*sin(q_1)*sin(q_2)*sin(q_3) - 1.0*cos(q_2)*cos(q_3)*sin(q_1)) + 0.0462*sin(q_1)*(1.0*cos(q_1)*cos(q_2)*cos(q_3) - 1.0*cos(q_1)*sin(q_2)*sin(q_3)))*(1.0*cos(q_1)*cos(q_2)*sin(q_3) + 1.0*cos(q_1)*cos(q_3)*sin(q_2)) - 1.0*(cos(q_1)*cos(q_2)*cos(q_3) - 1.0*cos(q_1)*sin(q_2)*sin(q_3))*(0.0016*cos(q_1)*(1.0*cos(q_2)*sin(q_1)*sin(q_3) + 1.0*cos(q_3)*sin(q_1)*sin(q_2)) - 0.0016*sin(q_1)*(cos(q_1)*cos(q_2)*sin(q_3) + 1.0*cos(q_1)*cos(q_3)*sin(q_2))) + (cos(q_1)*cos(q_2)*sin(q_3) + 1.0*cos(q_1)*cos(q_3)*sin(q_2))*(0.0016*cos(q_1)*(1.0*sin(q_1)*sin(q_2)*sin(q_3) - 1.0*cos(q_2)*cos(q_3)*sin(q_1)) + 0.0016*sin(q_1)*(cos(q_1)*cos(q_2)*cos(q_3) - 1.0*cos(q_1)*sin(q_2)*sin(q_3)))) + 4.55*cos(q_1)^2*(0.2723*cos(q_2)*cos(q_3) - 0.2723*sin(q_2)*sin(q_3))*(0.2723*cos(q_2)*sin(q_3) + 1.0*sin(q_2)*(0.2723*cos(q_3) + 0.425)) + 4.55*sin(q_1)^2*(0.2723*cos(q_2)*cos(q_3) - 0.2723*sin(q_2)*sin(q_3))*(0.2723*cos(q_2)*sin(q_3) + 1.0*sin(q_2)*(0.2723*cos(q_3) + 0.425))) + 0.5*dq_2*(1.0*cos(q_1)*((1.0*cos(q_2)*sin(q_1)*sin(q_3) + 1.0*cos(q_3)*sin(q_1)*sin(q_2))*(0.0016*cos(q_1)*(1.0*sin(q_1)*sin(q_2)*sin(q_3) - 1.0*cos(q_2)*cos(q_3)*sin(q_1)) + 0.0016*sin(q_1)*(cos(q_1)*cos(q_2)*cos(q_3) - 1.0*cos(q_1)*sin(q_2)*sin(q_3))) + (1.0*sin(q_1)*sin(q_2)*sin(q_3) - 1.0*cos(q_2)*cos(q_3)*sin(q_1))*(0.0016*cos(q_1)*(1.0*cos(q_2)*sin(q_1)*sin(q_3) + 1.0*cos(q_3)*sin(q_1)*sin(q_2)) - 0.0016*sin(q_1)*(1.0*cos(q_1)*cos(q_2)*sin(q_3) + cos(q_1)*cos(q_3)*sin(q_2))) - 1.0*(0.0462*cos(q_1)*(1.0*cos(q_2)*sin(q_1)*sin(q_3) + 1.0*cos(q_3)*sin(q_1)*sin(q_2)) - 0.0462*sin(q_1)*(1.0*cos(q_1)*cos(q_2)*sin(q_3) + 1.0*cos(q_1)*cos(q_3)*sin(q_2)))*(1.0*sin(q_1)*sin(q_2)*sin(q_3) - 1.0*cos(q_2)*cos(q_3)*sin(q_1)) - 1.0*(0.0462*cos(q_1)*(1.0*sin(q_1)*sin(q_2)*sin(q_3) - 1.0*cos(q_2)*cos(q_3)*sin(q_1)) + 0.0462*sin(q_1)*(1.0*cos(q_1)*cos(q_2)*cos(q_3) - 1.0*cos(q_1)*sin(q_2)*sin(q_3)))*(1.0*cos(q_2)*sin(q_1)*sin(q_3) + 1.0*cos(q_3)*sin(q_1)*sin(q_2))) - 0.758*cos(q_2)*sin(q_2) + (0.2723*cos(q_2)*sin(q_3) + 1.0*sin(q_2)*(0.2723*cos(q_3) + 0.425))*(0.6195*sin(q_2)*sin(q_3) - 2.275*cos(q_2)*(0.2723*cos(q_3) + 0.425)) + (0.2723*sin(q_2)*sin(q_3) - 1.0*cos(q_2)*(0.2723*cos(q_3) + 0.425))*(0.6195*cos(q_2)*sin(q_3) + 2.275*sin(q_2)*(0.2723*cos(q_3) + 0.425)) - 1.0*sin(q_1)*(1.0*(0.0462*cos(q_1)*(1.0*cos(q_2)*sin(q_1)*sin(q_3) + 1.0*cos(q_3)*sin(q_1)*sin(q_2)) - 0.0462*sin(q_1)*(1.0*cos(q_1)*cos(q_2)*sin(q_3) + 1.0*cos(q_1)*cos(q_3)*sin(q_2)))*(1.0*cos(q_1)*cos(q_2)*cos(q_3) - 1.0*cos(q_1)*sin(q_2)*sin(q_3)) - 1.0*(0.0462*cos(q_1)*(1.0*sin(q_1)*sin(q_2)*sin(q_3) - 1.0*cos(q_2)*cos(q_3)*sin(q_1)) + 0.0462*sin(q_1)*(1.0*cos(q_1)*cos(q_2)*cos(q_3) - 1.0*cos(q_1)*sin(q_2)*sin(q_3)))*(1.0*cos(q_1)*cos(q_2)*sin(q_3) + 1.0*cos(q_1)*cos(q_3)*sin(q_2)) - 1.0*(cos(q_1)*cos(q_2)*cos(q_3) - 1.0*cos(q_1)*sin(q_2)*sin(q_3))*(0.0016*cos(q_1)*(1.0*cos(q_2)*sin(q_1)*sin(q_3) + 1.0*cos(q_3)*sin(q_1)*sin(q_2)) - 0.0016*sin(q_1)*(1.0*cos(q_1)*cos(q_2)*sin(q_3) + cos(q_1)*cos(q_3)*sin(q_2))) + (1.0*cos(q_1)*cos(q_2)*sin(q_3) + cos(q_1)*cos(q_3)*sin(q_2))*(0.0016*cos(q_1)*(1.0*sin(q_1)*sin(q_2)*sin(q_3) - 1.0*cos(q_2)*cos(q_3)*sin(q_1)) + 0.0016*sin(q_1)*(cos(q_1)*cos(q_2)*cos(q_3) - 1.0*cos(q_1)*sin(q_2)*sin(q_3)))) + 0.758*cos(q_1)^2*cos(q_2)*sin(q_2) + 0.758*cos(q_2)*sin(q_1)^2*sin(q_2) - 4.55*cos(q_1)^2*(0.2723*cos(q_2)*sin(q_3) + 1.0*sin(q_2)*(0.2723*cos(q_3) + 0.425))*(0.2723*sin(q_2)*sin(q_3) - 1.0*cos(q_2)*(0.2723*cos(q_3) + 0.425)) - 4.55*sin(q_1)^2*(0.2723*cos(q_2)*sin(q_3) + 1.0*sin(q_2)*(0.2723*cos(q_3) + 0.425))*(0.2723*sin(q_2)*sin(q_3) - 1.0*cos(q_2)*(0.2723*cos(q_3) + 0.425))), 0.5*dq_1*(1.0*sin(q_1)*((1.0*sin(q_1)*sin(q_2)*sin(q_3) - 1.0*cos(q_2)*cos(q_3)*sin(q_1))*(0.0016*cos(q_1)*(1.0*sin(q_1)*sin(q_2)*sin(q_3) - 1.0*cos(q_2)*cos(q_3)*sin(q_1)) + 0.0016*sin(q_1)*(cos(q_1)*cos(q_2)*cos(q_3) - 1.0*cos(q_1)*sin(q_2)*sin(q_3))) + 1.0*(0.0462*cos(q_1)*(1.0*cos(q_2)*sin(q_1)*sin(q_3) + 1.0*cos(q_3)*sin(q_1)*sin(q_2)) - 0.0462*sin(q_1)*(1.0*cos(q_1)*cos(q_2)*sin(q_3) + 1.0*cos(q_1)*cos(q_3)*sin(q_2)))*(1.0*cos(q_2)*sin(q_1)*sin(q_3) + 1.0*cos(q_3)*sin(q_1)*sin(q_2)) + 1.0*cos(q_1)*(0.0462*cos(q_1)^2 + 0.0462*sin(q_1)^2) + 1.0*(cos(q_1)*cos(q_2)*cos(q_3) - 1.0*cos(q_1)*sin(q_2)*sin(q_3))*(0.0016*cos(q_1)*(cos(q_1)*cos(q_2)*cos(q_3) - 1.0*cos(q_1)*sin(q_2)*sin(q_3)) - 0.0016*cos(q_1)*(1.0*cos(q_1)*cos(q_2)*cos(q_3) - 1.0*cos(q_1)*sin(q_2)*sin(q_3)))) - 1.0*sin(q_1)*((1.0*sin(q_1)*sin(q_2)*sin(q_3) - 1.0*cos(q_2)*cos(q_3)*sin(q_1))*(0.0016*cos(q_1)*(1.0*sin(q_1)*sin(q_2)*sin(q_3) - 1.0*cos(q_2)*cos(q_3)*sin(q_1)) + 0.0016*sin(q_1)*(cos(q_1)*cos(q_2)*cos(q_3) - 1.0*cos(q_1)*sin(q_2)*sin(q_3))) + (0.0462*cos(q_1)*(1.0*cos(q_2)*sin(q_1)*sin(q_3) + 1.0*cos(q_3)*sin(q_1)*sin(q_2)) - 0.0462*sin(q_1)*(1.0*cos(q_1)*cos(q_2)*sin(q_3) + 1.0*cos(q_1)*cos(q_3)*sin(q_2)))*(1.0*cos(q_2)*sin(q_1)*sin(q_3) + 1.0*cos(q_3)*sin(q_1)*sin(q_2)) + 1.0*cos(q_1)*(0.0462*cos(q_1)^2 + 0.0462*sin(q_1)^2)) + 1.0*cos(q_1)*((0.0016*cos(q_1)*(cos(q_1)*cos(q_2)*cos(q_3) - 1.0*cos(q_1)*sin(q_2)*sin(q_3)) - 0.0016*cos(q_1)*(1.0*cos(q_1)*cos(q_2)*cos(q_3) - 1.0*cos(q_1)*sin(q_2)*sin(q_3)))*(1.0*sin(q_1)*sin(q_2)*sin(q_3) - 1.0*cos(q_2)*cos(q_3)*sin(q_1)) - 1.0*(1.0*cos(q_1)*cos(q_2)*cos(q_3) - 1.0*cos(q_1)*sin(q_2)*sin(q_3))*(0.0016*cos(q_1)*(1.0*sin(q_1)*sin(q_2)*sin(q_3) - 1.0*cos(q_2)*cos(q_3)*sin(q_1)) + 0.0016*sin(q_1)*(cos(q_1)*cos(q_2)*cos(q_3) - 1.0*cos(q_1)*sin(q_2)*sin(q_3))) + 1.0*(0.0462*cos(q_1)*(1.0*cos(q_2)*sin(q_1)*sin(q_3) + 1.0*cos(q_3)*sin(q_1)*sin(q_2)) - 0.0462*sin(q_1)*(1.0*cos(q_1)*cos(q_2)*sin(q_3) + 1.0*cos(q_1)*cos(q_3)*sin(q_2)))*(1.0*cos(q_1)*cos(q_2)*sin(q_3) + 1.0*cos(q_1)*cos(q_3)*sin(q_2)) - 1.0*sin(q_1)*(0.0462*cos(q_1)^2 + 0.0462*sin(q_1)^2)) + 1.0*cos(q_1)*((0.0462*cos(q_2)*cos(q_3) - 0.0462*sin(q_2)*sin(q_3))*(1.0*sin(q_1)*sin(q_2)*sin(q_3) - 1.0*cos(q_2)*cos(q_3)*sin(q_1)) + (0.0462*cos(q_2)*sin(q_3) + 0.0462*cos(q_3)*sin(q_2))*(1.0*cos(q_2)*sin(q_1)*sin(q_3) + 1.0*cos(q_3)*sin(q_1)*sin(q_2)) - 1.0*(0.0016*cos(q_2)*cos(q_3) - 0.0016*sin(q_2)*sin(q_3))*(1.0*sin(q_1)*sin(q_2)*sin(q_3) - 1.0*cos(q_2)*cos(q_3)*sin(q_1)) - 1.0*(0.0016*cos(q_2)*sin(q_3) + 0.0016*cos(q_3)*sin(q_2))*(1.0*cos(q_2)*sin(q_1)*sin(q_3) + 1.0*cos(q_3)*sin(q_1)*sin(q_2))) + 1.0*(1.0*cos(q_2)*cos(q_3) - 1.0*sin(q_2)*sin(q_3))*(0.0016*cos(q_1)*(1.0*sin(q_1)*sin(q_2)*sin(q_3) - 1.0*cos(q_2)*cos(q_3)*sin(q_1)) + 0.0016*sin(q_1)*(cos(q_1)*cos(q_2)*cos(q_3) - 1.0*cos(q_1)*sin(q_2)*sin(q_3))) + 1.0*(1.0*cos(q_2)*sin(q_3) + 1.0*cos(q_3)*sin(q_2))*(0.0016*cos(q_1)*(1.0*cos(q_2)*sin(q_1)*sin(q_3) + 1.0*cos(q_3)*sin(q_1)*sin(q_2)) - 0.0016*sin(q_1)*(cos(q_1)*cos(q_2)*sin(q_3) + 1.0*cos(q_1)*cos(q_3)*sin(q_2))) - 1.0*(1.0*cos(q_2)*cos(q_3) - 1.0*sin(q_2)*sin(q_3))*(0.0462*cos(q_1)*(1.0*sin(q_1)*sin(q_2)*sin(q_3) - 1.0*cos(q_2)*cos(q_3)*sin(q_1)) + 0.0462*sin(q_1)*(1.0*cos(q_1)*cos(q_2)*cos(q_3) - 1.0*cos(q_1)*sin(q_2)*sin(q_3))) - 1.0*(1.0*cos(q_2)*sin(q_3) + 1.0*cos(q_3)*sin(q_2))*(0.0462*cos(q_1)*(1.0*cos(q_2)*sin(q_1)*sin(q_3) + 1.0*cos(q_3)*sin(q_1)*sin(q_2)) - 0.0462*sin(q_1)*(1.0*cos(q_1)*cos(q_2)*sin(q_3) + 1.0*cos(q_1)*cos(q_3)*sin(q_2))) - 1.0*sin(q_1)*((0.0016*cos(q_2)*cos(q_3) - 0.0016*sin(q_2)*sin(q_3))*(cos(q_1)*cos(q_2)*cos(q_3) - 1.0*cos(q_1)*sin(q_2)*sin(q_3)) - 1.0*(0.0016*cos(q_2)*sin(q_3) + 0.0016*cos(q_3)*sin(q_2))*(1.0*cos(q_1)*cos(q_2)*sin(q_3) + cos(q_1)*cos(q_3)*sin(q_2)) - 1.0*(0.0462*cos(q_2)*cos(q_3) - 0.0462*sin(q_2)*sin(q_3))*(1.0*cos(q_1)*cos(q_2)*cos(q_3) - 1.0*cos(q_1)*sin(q_2)*sin(q_3)) + 1.0*(0.0462*cos(q_2)*sin(q_3) + 0.0462*cos(q_3)*sin(q_2))*(1.0*cos(q_1)*cos(q_2)*sin(q_3) + 1.0*cos(q_1)*cos(q_3)*sin(q_2))) + 1.0*cos(q_1)*(1.0*sin(q_1)*(0.0462*cos(q_1)^2 + 0.0462*sin(q_1)^2) - 1.0*(0.0462*cos(q_1)*(1.0*cos(q_2)*sin(q_1)*sin(q_3) + 1.0*cos(q_3)*sin(q_1)*sin(q_2)) - 0.0462*sin(q_1)*(1.0*cos(q_1)*cos(q_2)*sin(q_3) + 1.0*cos(q_1)*cos(q_3)*sin(q_2)))*(1.0*cos(q_1)*cos(q_2)*sin(q_3) + 1.0*cos(q_1)*cos(q_3)*sin(q_2)) + (cos(q_1)*cos(q_2)*cos(q_3) - 1.0*cos(q_1)*sin(q_2)*sin(q_3))*(0.0016*cos(q_1)*(1.0*sin(q_1)*sin(q_2)*sin(q_3) - 1.0*cos(q_2)*cos(q_3)*sin(q_1)) + 0.0016*sin(q_1)*(cos(q_1)*cos(q_2)*cos(q_3) - 1.0*cos(q_1)*sin(q_2)*sin(q_3)))) - 2.275*cos(q_1)*(0.0265*cos(q_1) + 1.0*sin(q_1)*(0.2723*sin(q_2)*sin(q_3) - 1.0*cos(q_2)*(0.2723*cos(q_3) + 0.425)))*(0.2723*cos(q_2)*cos(q_3) - 0.2723*sin(q_2)*sin(q_3)) - 2.275*sin(q_1)*(0.0265*sin(q_1) - 1.0*cos(q_1)*(0.2723*sin(q_2)*sin(q_3) - 1.0*cos(q_2)*(0.2723*cos(q_3) + 0.425)))*(0.2723*cos(q_2)*cos(q_3) - 0.2723*sin(q_2)*sin(q_3)) + 1.0*cos(q_1)*(0.2723*cos(q_2)*cos(q_3) - 0.2723*sin(q_2)*sin(q_3))*(0.06029*cos(q_1) + 2.275*sin(q_1)*(0.2723*sin(q_2)*sin(q_3) - 1.0*cos(q_2)*(0.2723*cos(q_3) + 0.425))) + 1.0*sin(q_1)*(0.2723*cos(q_2)*cos(q_3) - 0.2723*sin(q_2)*sin(q_3))*(0.06029*sin(q_1) - 2.275*cos(q_1)*(0.2723*sin(q_2)*sin(q_3) - 1.0*cos(q_2)*(0.2723*cos(q_3) + 0.425)))) + 0.5*dq_2*(1.0*(0.2723*cos(q_2)*sin(q_3) + 0.2723*cos(q_3)*sin(q_2))*(0.6195*sin(q_2)*sin(q_3) - 2.275*cos(q_2)*(0.2723*cos(q_3) + 0.425)) + (0.6195*cos(q_2)*sin(q_3) + 0.6195*cos(q_3)*sin(q_2))*(0.2723*sin(q_2)*sin(q_3) - 1.0*cos(q_2)*(0.2723*cos(q_3) + 0.425)) + 1.0*cos(q_1)*((1.0*cos(q_2)*sin(q_1)*sin(q_3) + 1.0*cos(q_3)*sin(q_1)*sin(q_2))*(0.0016*cos(q_1)*(1.0*sin(q_1)*sin(q_2)*sin(q_3) - 1.0*cos(q_2)*cos(q_3)*sin(q_1)) + 0.0016*sin(q_1)*(cos(q_1)*cos(q_2)*cos(q_3) - 1.0*cos(q_1)*sin(q_2)*sin(q_3))) + (1.0*sin(q_1)*sin(q_2)*sin(q_3) - 1.0*cos(q_2)*cos(q_3)*sin(q_1))*(0.0016*cos(q_1)*(1.0*cos(q_2)*sin(q_1)*sin(q_3) + 1.0*cos(q_3)*sin(q_1)*sin(q_2)) - 0.0016*sin(q_1)*(cos(q_1)*cos(q_2)*sin(q_3) + 1.0*cos(q_1)*cos(q_3)*sin(q_2))) - 1.0*(0.0462*cos(q_1)*(1.0*cos(q_2)*sin(q_1)*sin(q_3) + 1.0*cos(q_3)*sin(q_1)*sin(q_2)) - 0.0462*sin(q_1)*(1.0*cos(q_1)*cos(q_2)*sin(q_3) + 1.0*cos(q_1)*cos(q_3)*sin(q_2)))*(1.0*sin(q_1)*sin(q_2)*sin(q_3) - 1.0*cos(q_2)*cos(q_3)*sin(q_1)) - 1.0*(0.0462*cos(q_1)*(1.0*sin(q_1)*sin(q_2)*sin(q_3) - 1.0*cos(q_2)*cos(q_3)*sin(q_1)) + 0.0462*sin(q_1)*(1.0*cos(q_1)*cos(q_2)*cos(q_3) - 1.0*cos(q_1)*sin(q_2)*sin(q_3)))*(1.0*cos(q_2)*sin(q_1)*sin(q_3) + 1.0*cos(q_3)*sin(q_1)*sin(q_2))) - 1.0*sin(q_1)*(1.0*(0.0462*cos(q_1)*(1.0*cos(q_2)*sin(q_1)*sin(q_3) + 1.0*cos(q_3)*sin(q_1)*sin(q_2)) - 0.0462*sin(q_1)*(1.0*cos(q_1)*cos(q_2)*sin(q_3) + 1.0*cos(q_1)*cos(q_3)*sin(q_2)))*(1.0*cos(q_1)*cos(q_2)*cos(q_3) - 1.0*cos(q_1)*sin(q_2)*sin(q_3)) - 1.0*(0.0462*cos(q_1)*(1.0*sin(q_1)*sin(q_2)*sin(q_3) - 1.0*cos(q_2)*cos(q_3)*sin(q_1)) + 0.0462*sin(q_1)*(1.0*cos(q_1)*cos(q_2)*cos(q_3) - 1.0*cos(q_1)*sin(q_2)*sin(q_3)))*(1.0*cos(q_1)*cos(q_2)*sin(q_3) + 1.0*cos(q_1)*cos(q_3)*sin(q_2)) - 1.0*(cos(q_1)*cos(q_2)*cos(q_3) - 1.0*cos(q_1)*sin(q_2)*sin(q_3))*(0.0016*cos(q_1)*(1.0*cos(q_2)*sin(q_1)*sin(q_3) + 1.0*cos(q_3)*sin(q_1)*sin(q_2)) - 0.0016*sin(q_1)*(cos(q_1)*cos(q_2)*sin(q_3) + 1.0*cos(q_1)*cos(q_3)*sin(q_2))) + (cos(q_1)*cos(q_2)*sin(q_3) + 1.0*cos(q_1)*cos(q_3)*sin(q_2))*(0.0016*cos(q_1)*(1.0*sin(q_1)*sin(q_2)*sin(q_3) - 1.0*cos(q_2)*cos(q_3)*sin(q_1)) + 0.0016*sin(q_1)*(cos(q_1)*cos(q_2)*cos(q_3) - 1.0*cos(q_1)*sin(q_2)*sin(q_3)))) + 4.55*cos(q_1)^2*(0.2723*cos(q_2)*cos(q_3) - 0.2723*sin(q_2)*sin(q_3))*(0.2723*cos(q_2)*sin(q_3) + 1.0*sin(q_2)*(0.2723*cos(q_3) + 0.425)) + 4.55*sin(q_1)^2*(0.2723*cos(q_2)*cos(q_3) - 0.2723*sin(q_2)*sin(q_3))*(0.2723*cos(q_2)*sin(q_3) + 1.0*sin(q_2)*(0.2723*cos(q_3) + 0.425))) + 0.5*dq_3*(2.0*(0.2723*cos(q_2)*sin(q_3) + 0.2723*cos(q_3)*sin(q_2))*(0.6195*sin(q_2)*sin(q_3) - 2.275*cos(q_2)*(0.2723*cos(q_3) + 0.425)) + 2.0*cos(q_1)*((1.0*cos(q_2)*sin(q_1)*sin(q_3) + 1.0*cos(q_3)*sin(q_1)*sin(q_2))*(0.0016*cos(q_1)*(1.0*sin(q_1)*sin(q_2)*sin(q_3) - 1.0*cos(q_2)*cos(q_3)*sin(q_1)) + 0.0016*sin(q_1)*(cos(q_1)*cos(q_2)*cos(q_3) - 1.0*cos(q_1)*sin(q_2)*sin(q_3))) + (1.0*sin(q_1)*sin(q_2)*sin(q_3) - 1.0*cos(q_2)*cos(q_3)*sin(q_1))*(0.0016*cos(q_1)*(1.0*cos(q_2)*sin(q_1)*sin(q_3) + 1.0*cos(q_3)*sin(q_1)*sin(q_2)) - 0.0016*sin(q_1)*(cos(q_1)*cos(q_2)*sin(q_3) + 1.0*cos(q_1)*cos(q_3)*sin(q_2))) - 1.0*(0.0462*cos(q_1)*(1.0*cos(q_2)*sin(q_1)*sin(q_3) + 1.0*cos(q_3)*sin(q_1)*sin(q_2)) - 0.0462*sin(q_1)*(1.0*cos(q_1)*cos(q_2)*sin(q_3) + 1.0*cos(q_1)*cos(q_3)*sin(q_2)))*(1.0*sin(q_1)*sin(q_2)*sin(q_3) - 1.0*cos(q_2)*cos(q_3)*sin(q_1)) - 1.0*(0.0462*cos(q_1)*(1.0*sin(q_1)*sin(q_2)*sin(q_3) - 1.0*cos(q_2)*cos(q_3)*sin(q_1)) + 0.0462*sin(q_1)*(1.0*cos(q_1)*cos(q_2)*cos(q_3) - 1.0*cos(q_1)*sin(q_2)*sin(q_3)))*(1.0*cos(q_2)*sin(q_1)*sin(q_3) + 1.0*cos(q_3)*sin(q_1)*sin(q_2))) - 1.0*cos(q_1)*((1.0*cos(q_2)*sin(q_1)*sin(q_3) + 1.0*cos(q_3)*sin(q_1)*sin(q_2))*(0.0016*cos(q_1)*(1.0*sin(q_1)*sin(q_2)*sin(q_3) - 1.0*cos(q_2)*cos(q_3)*sin(q_1)) + 0.0016*sin(q_1)*(cos(q_1)*cos(q_2)*cos(q_3) - 1.0*cos(q_1)*sin(q_2)*sin(q_3))) + (1.0*sin(q_1)*sin(q_2)*sin(q_3) - 1.0*cos(q_2)*cos(q_3)*sin(q_1))*(0.0016*cos(q_1)*(1.0*cos(q_2)*sin(q_1)*sin(q_3) + 1.0*cos(q_3)*sin(q_1)*sin(q_2)) - 0.0016*sin(q_1)*(1.0*cos(q_1)*cos(q_2)*sin(q_3) + cos(q_1)*cos(q_3)*sin(q_2))) - 1.0*(0.0462*cos(q_1)*(1.0*cos(q_2)*sin(q_1)*sin(q_3) + 1.0*cos(q_3)*sin(q_1)*sin(q_2)) - 0.0462*sin(q_1)*(1.0*cos(q_1)*cos(q_2)*sin(q_3) + 1.0*cos(q_1)*cos(q_3)*sin(q_2)))*(1.0*sin(q_1)*sin(q_2)*sin(q_3) - 1.0*cos(q_2)*cos(q_3)*sin(q_1)) - 1.0*(0.0462*cos(q_1)*(1.0*sin(q_1)*sin(q_2)*sin(q_3) - 1.0*cos(q_2)*cos(q_3)*sin(q_1)) + 0.0462*sin(q_1)*(1.0*cos(q_1)*cos(q_2)*cos(q_3) - 1.0*cos(q_1)*sin(q_2)*sin(q_3)))*(1.0*cos(q_2)*sin(q_1)*sin(q_3) + 1.0*cos(q_3)*sin(q_1)*sin(q_2))) - 2.0*sin(q_1)*(1.0*(0.0462*cos(q_1)*(1.0*cos(q_2)*sin(q_1)*sin(q_3) + 1.0*cos(q_3)*sin(q_1)*sin(q_2)) - 0.0462*sin(q_1)*(1.0*cos(q_1)*cos(q_2)*sin(q_3) + 1.0*cos(q_1)*cos(q_3)*sin(q_2)))*(1.0*cos(q_1)*cos(q_2)*cos(q_3) - 1.0*cos(q_1)*sin(q_2)*sin(q_3)) - 1.0*(0.0462*cos(q_1)*(1.0*sin(q_1)*sin(q_2)*sin(q_3) - 1.0*cos(q_2)*cos(q_3)*sin(q_1)) + 0.0462*sin(q_1)*(1.0*cos(q_1)*cos(q_2)*cos(q_3) - 1.0*cos(q_1)*sin(q_2)*sin(q_3)))*(1.0*cos(q_1)*cos(q_2)*sin(q_3) + 1.0*cos(q_1)*cos(q_3)*sin(q_2)) - 1.0*(cos(q_1)*cos(q_2)*cos(q_3) - 1.0*cos(q_1)*sin(q_2)*sin(q_3))*(0.0016*cos(q_1)*(1.0*cos(q_2)*sin(q_1)*sin(q_3) + 1.0*cos(q_3)*sin(q_1)*sin(q_2)) - 0.0016*sin(q_1)*(cos(q_1)*cos(q_2)*sin(q_3) + 1.0*cos(q_1)*cos(q_3)*sin(q_2))) + (cos(q_1)*cos(q_2)*sin(q_3) + 1.0*cos(q_1)*cos(q_3)*sin(q_2))*(0.0016*cos(q_1)*(1.0*sin(q_1)*sin(q_2)*sin(q_3) - 1.0*cos(q_2)*cos(q_3)*sin(q_1)) + 0.0016*sin(q_1)*(cos(q_1)*cos(q_2)*cos(q_3) - 1.0*cos(q_1)*sin(q_2)*sin(q_3)))) + 1.0*sin(q_1)*(1.0*(0.0462*cos(q_1)*(1.0*cos(q_2)*sin(q_1)*sin(q_3) + 1.0*cos(q_3)*sin(q_1)*sin(q_2)) - 0.0462*sin(q_1)*(1.0*cos(q_1)*cos(q_2)*sin(q_3) + 1.0*cos(q_1)*cos(q_3)*sin(q_2)))*(1.0*cos(q_1)*cos(q_2)*cos(q_3) - 1.0*cos(q_1)*sin(q_2)*sin(q_3)) - 1.0*(0.0462*cos(q_1)*(1.0*sin(q_1)*sin(q_2)*sin(q_3) - 1.0*cos(q_2)*cos(q_3)*sin(q_1)) + 0.0462*sin(q_1)*(1.0*cos(q_1)*cos(q_2)*cos(q_3) - 1.0*cos(q_1)*sin(q_2)*sin(q_3)))*(1.0*cos(q_1)*cos(q_2)*sin(q_3) + 1.0*cos(q_1)*cos(q_3)*sin(q_2)) - 1.0*(cos(q_1)*cos(q_2)*cos(q_3) - 1.0*cos(q_1)*sin(q_2)*sin(q_3))*(0.0016*cos(q_1)*(1.0*cos(q_2)*sin(q_1)*sin(q_3) + 1.0*cos(q_3)*sin(q_1)*sin(q_2)) - 0.0016*sin(q_1)*(1.0*cos(q_1)*cos(q_2)*sin(q_3) + cos(q_1)*cos(q_3)*sin(q_2))) + (1.0*cos(q_1)*cos(q_2)*sin(q_3) + cos(q_1)*cos(q_3)*sin(q_2))*(0.0016*cos(q_1)*(1.0*sin(q_1)*sin(q_2)*sin(q_3) - 1.0*cos(q_2)*cos(q_3)*sin(q_1)) + 0.0016*sin(q_1)*(cos(q_1)*cos(q_2)*cos(q_3) - 1.0*cos(q_1)*sin(q_2)*sin(q_3)))) + (0.2723*cos(q_2)*cos(q_3) - 0.2723*sin(q_2)*sin(q_3))*(0.6195*cos(q_2)*sin(q_3) + 0.6195*cos(q_3)*sin(q_2)) - 2.0*(0.2723*cos(q_2)*cos(q_3) - 0.2723*sin(q_2)*sin(q_3))*(0.6195*cos(q_2)*sin(q_3) + 0.6195*cos(q_3)*sin(q_2)) + (0.2723*cos(q_2)*sin(q_3) + 0.2723*cos(q_3)*sin(q_2))*(0.6195*cos(q_2)*cos(q_3) - 0.6195*sin(q_2)*sin(q_3)) + 4.55*cos(q_1)^2*(0.2723*cos(q_2)*cos(q_3) - 0.2723*sin(q_2)*sin(q_3))*(0.2723*cos(q_2)*sin(q_3) + 1.0*sin(q_2)*(0.2723*cos(q_3) + 0.425)) + 4.55*sin(q_1)^2*(0.2723*cos(q_2)*cos(q_3) - 0.2723*sin(q_2)*sin(q_3))*(0.2723*cos(q_2)*sin(q_3) + 1.0*sin(q_2)*(0.2723*cos(q_3) + 0.425)));
                                                                                                                                                                                                                                                                                                                                                                               0.5*dq_3*(1.0*sin(q_1)*((1.0*sin(q_1)*sin(q_2)*sin(q_3) - 1.0*cos(q_2)*cos(q_3)*sin(q_1))*(0.0016*cos(q_1)*(1.0*sin(q_1)*sin(q_2)*sin(q_3) - 1.0*cos(q_2)*cos(q_3)*sin(q_1)) + 0.0016*sin(q_1)*(cos(q_1)*cos(q_2)*cos(q_3) - 1.0*cos(q_1)*sin(q_2)*sin(q_3))) + 1.0*(0.0462*cos(q_1)*(1.0*cos(q_2)*sin(q_1)*sin(q_3) + 1.0*cos(q_3)*sin(q_1)*sin(q_2)) - 0.0462*sin(q_1)*(1.0*cos(q_1)*cos(q_2)*sin(q_3) + 1.0*cos(q_1)*cos(q_3)*sin(q_2)))*(1.0*cos(q_2)*sin(q_1)*sin(q_3) + 1.0*cos(q_3)*sin(q_1)*sin(q_2)) + 1.0*cos(q_1)*(0.0462*cos(q_1)^2 + 0.0462*sin(q_1)^2) + 1.0*(cos(q_1)*cos(q_2)*cos(q_3) - 1.0*cos(q_1)*sin(q_2)*sin(q_3))*(0.0016*cos(q_1)*(cos(q_1)*cos(q_2)*cos(q_3) - 1.0*cos(q_1)*sin(q_2)*sin(q_3)) - 0.0016*cos(q_1)*(1.0*cos(q_1)*cos(q_2)*cos(q_3) - 1.0*cos(q_1)*sin(q_2)*sin(q_3)))) - 1.0*sin(q_1)*((1.0*sin(q_1)*sin(q_2)*sin(q_3) - 1.0*cos(q_2)*cos(q_3)*sin(q_1))*(0.0016*cos(q_1)*(1.0*sin(q_1)*sin(q_2)*sin(q_3) - 1.0*cos(q_2)*cos(q_3)*sin(q_1)) + 0.0016*sin(q_1)*(cos(q_1)*cos(q_2)*cos(q_3) - 1.0*cos(q_1)*sin(q_2)*sin(q_3))) + (0.0462*cos(q_1)*(1.0*cos(q_2)*sin(q_1)*sin(q_3) + 1.0*cos(q_3)*sin(q_1)*sin(q_2)) - 0.0462*sin(q_1)*(1.0*cos(q_1)*cos(q_2)*sin(q_3) + 1.0*cos(q_1)*cos(q_3)*sin(q_2)))*(1.0*cos(q_2)*sin(q_1)*sin(q_3) + 1.0*cos(q_3)*sin(q_1)*sin(q_2)) + 1.0*cos(q_1)*(0.0462*cos(q_1)^2 + 0.0462*sin(q_1)^2)) + 1.0*cos(q_1)*((0.0016*cos(q_1)*(cos(q_1)*cos(q_2)*cos(q_3) - 1.0*cos(q_1)*sin(q_2)*sin(q_3)) - 0.0016*cos(q_1)*(1.0*cos(q_1)*cos(q_2)*cos(q_3) - 1.0*cos(q_1)*sin(q_2)*sin(q_3)))*(1.0*sin(q_1)*sin(q_2)*sin(q_3) - 1.0*cos(q_2)*cos(q_3)*sin(q_1)) - 1.0*(1.0*cos(q_1)*cos(q_2)*cos(q_3) - 1.0*cos(q_1)*sin(q_2)*sin(q_3))*(0.0016*cos(q_1)*(1.0*sin(q_1)*sin(q_2)*sin(q_3) - 1.0*cos(q_2)*cos(q_3)*sin(q_1)) + 0.0016*sin(q_1)*(cos(q_1)*cos(q_2)*cos(q_3) - 1.0*cos(q_1)*sin(q_2)*sin(q_3))) + 1.0*(0.0462*cos(q_1)*(1.0*cos(q_2)*sin(q_1)*sin(q_3) + 1.0*cos(q_3)*sin(q_1)*sin(q_2)) - 0.0462*sin(q_1)*(1.0*cos(q_1)*cos(q_2)*sin(q_3) + 1.0*cos(q_1)*cos(q_3)*sin(q_2)))*(1.0*cos(q_1)*cos(q_2)*sin(q_3) + 1.0*cos(q_1)*cos(q_3)*sin(q_2)) - 1.0*sin(q_1)*(0.0462*cos(q_1)^2 + 0.0462*sin(q_1)^2)) + 1.0*cos(q_1)*(1.0*sin(q_1)*(0.0462*cos(q_1)^2 + 0.0462*sin(q_1)^2) - 1.0*(0.0462*cos(q_1)*(1.0*cos(q_2)*sin(q_1)*sin(q_3) + 1.0*cos(q_3)*sin(q_1)*sin(q_2)) - 0.0462*sin(q_1)*(1.0*cos(q_1)*cos(q_2)*sin(q_3) + 1.0*cos(q_1)*cos(q_3)*sin(q_2)))*(1.0*cos(q_1)*cos(q_2)*sin(q_3) + 1.0*cos(q_1)*cos(q_3)*sin(q_2)) + (cos(q_1)*cos(q_2)*cos(q_3) - 1.0*cos(q_1)*sin(q_2)*sin(q_3))*(0.0016*cos(q_1)*(1.0*sin(q_1)*sin(q_2)*sin(q_3) - 1.0*cos(q_2)*cos(q_3)*sin(q_1)) + 0.0016*sin(q_1)*(cos(q_1)*cos(q_2)*cos(q_3) - 1.0*cos(q_1)*sin(q_2)*sin(q_3))))) + 0.5*dq_1*(2.0*(1.0*cos(q_2)*sin(q_3) + 1.0*cos(q_3)*sin(q_2))*(0.0016*cos(q_1)*(cos(q_1)*cos(q_2)*cos(q_3) - 1.0*cos(q_1)*sin(q_2)*sin(q_3)) - 0.0016*cos(q_1)*(1.0*cos(q_1)*cos(q_2)*cos(q_3) - 1.0*cos(q_1)*sin(q_2)*sin(q_3))) + 1.0*(1.0*cos(q_2)*cos(q_3) - 1.0*sin(q_2)*sin(q_3))*(0.0462*cos(q_2)*sin(q_3) + 0.0462*cos(q_3)*sin(q_2)) + 1.0*(1.0*cos(q_2)*sin(q_3) + 1.0*cos(q_3)*sin(q_2))*(0.0462*cos(q_2)*cos(q_3) - 0.0462*sin(q_2)*sin(q_3)) - 1.0*(1.0*cos(q_2)*cos(q_3) - 1.0*sin(q_2)*sin(q_3))*(0.0016*cos(q_2)*sin(q_3) + 0.0016*cos(q_3)*sin(q_2)) - 1.0*(1.0*cos(q_2)*sin(q_3) + 1.0*cos(q_3)*sin(q_2))*(0.0016*cos(q_2)*cos(q_3) - 0.0016*sin(q_2)*sin(q_3)) + 2.275*cos(q_1)*(0.0265*sin(q_1) - 1.0*cos(q_1)*(0.2723*sin(q_2)*sin(q_3) - 1.0*cos(q_2)*(0.2723*cos(q_3) + 0.425)))*(0.2723*cos(q_2)*sin(q_3) + 0.2723*cos(q_3)*sin(q_2)) - 2.275*sin(q_1)*(0.0265*cos(q_1) + 1.0*sin(q_1)*(0.2723*sin(q_2)*sin(q_3) - 1.0*cos(q_2)*(0.2723*cos(q_3) + 0.425)))*(0.2723*cos(q_2)*sin(q_3) + 0.2723*cos(q_3)*sin(q_2)) + 1.0*cos(q_1)*(0.2723*cos(q_2)*sin(q_3) + 0.2723*cos(q_3)*sin(q_2))*(0.06029*sin(q_1) - 2.275*cos(q_1)*(0.2723*sin(q_2)*sin(q_3) - 1.0*cos(q_2)*(0.2723*cos(q_3) + 0.425))) - 1.0*sin(q_1)*(0.2723*cos(q_2)*sin(q_3) + 0.2723*cos(q_3)*sin(q_2))*(0.06029*cos(q_1) + 2.275*sin(q_1)*(0.2723*sin(q_2)*sin(q_3) - 1.0*cos(q_2)*(0.2723*cos(q_3) + 0.425)))) + 0.5*dq_2*(1.0*sin(q_1)*((1.0*sin(q_1)*sin(q_2)*sin(q_3) - 1.0*cos(q_2)*cos(q_3)*sin(q_1))*(0.0016*cos(q_1)*(1.0*sin(q_1)*sin(q_2)*sin(q_3) - 1.0*cos(q_2)*cos(q_3)*sin(q_1)) + 0.0016*sin(q_1)*(cos(q_1)*cos(q_2)*cos(q_3) - 1.0*cos(q_1)*sin(q_2)*sin(q_3))) + 1.0*(0.0462*cos(q_1)*(1.0*cos(q_2)*sin(q_1)*sin(q_3) + 1.0*cos(q_3)*sin(q_1)*sin(q_2)) - 0.0462*sin(q_1)*(1.0*cos(q_1)*cos(q_2)*sin(q_3) + 1.0*cos(q_1)*cos(q_3)*sin(q_2)))*(1.0*cos(q_2)*sin(q_1)*sin(q_3) + 1.0*cos(q_3)*sin(q_1)*sin(q_2)) + 1.0*cos(q_1)*(0.0462*cos(q_1)^2 + 0.0462*sin(q_1)^2) + 1.0*(cos(q_1)*cos(q_2)*cos(q_3) - 1.0*cos(q_1)*sin(q_2)*sin(q_3))*(0.0016*cos(q_1)*(cos(q_1)*cos(q_2)*cos(q_3) - 1.0*cos(q_1)*sin(q_2)*sin(q_3)) - 0.0016*cos(q_1)*(1.0*cos(q_1)*cos(q_2)*cos(q_3) - 1.0*cos(q_1)*sin(q_2)*sin(q_3)))) - 1.0*sin(q_1)*((1.0*sin(q_1)*sin(q_2)*sin(q_3) - 1.0*cos(q_2)*cos(q_3)*sin(q_1))*(0.0016*cos(q_1)*(1.0*sin(q_1)*sin(q_2)*sin(q_3) - 1.0*cos(q_2)*cos(q_3)*sin(q_1)) + 0.0016*sin(q_1)*(cos(q_1)*cos(q_2)*cos(q_3) - 1.0*cos(q_1)*sin(q_2)*sin(q_3))) + (0.0462*cos(q_1)*(1.0*cos(q_2)*sin(q_1)*sin(q_3) + 1.0*cos(q_3)*sin(q_1)*sin(q_2)) - 0.0462*sin(q_1)*(1.0*cos(q_1)*cos(q_2)*sin(q_3) + 1.0*cos(q_1)*cos(q_3)*sin(q_2)))*(1.0*cos(q_2)*sin(q_1)*sin(q_3) + 1.0*cos(q_3)*sin(q_1)*sin(q_2)) + 1.0*cos(q_1)*(0.0462*cos(q_1)^2 + 0.0462*sin(q_1)^2)) + 1.0*cos(q_1)*((0.0016*cos(q_1)*(cos(q_1)*cos(q_2)*cos(q_3) - 1.0*cos(q_1)*sin(q_2)*sin(q_3)) - 0.0016*cos(q_1)*(1.0*cos(q_1)*cos(q_2)*cos(q_3) - 1.0*cos(q_1)*sin(q_2)*sin(q_3)))*(1.0*sin(q_1)*sin(q_2)*sin(q_3) - 1.0*cos(q_2)*cos(q_3)*sin(q_1)) - 1.0*(1.0*cos(q_1)*cos(q_2)*cos(q_3) - 1.0*cos(q_1)*sin(q_2)*sin(q_3))*(0.0016*cos(q_1)*(1.0*sin(q_1)*sin(q_2)*sin(q_3) - 1.0*cos(q_2)*cos(q_3)*sin(q_1)) + 0.0016*sin(q_1)*(cos(q_1)*cos(q_2)*cos(q_3) - 1.0*cos(q_1)*sin(q_2)*sin(q_3))) + 1.0*(0.0462*cos(q_1)*(1.0*cos(q_2)*sin(q_1)*sin(q_3) + 1.0*cos(q_3)*sin(q_1)*sin(q_2)) - 0.0462*sin(q_1)*(1.0*cos(q_1)*cos(q_2)*sin(q_3) + 1.0*cos(q_1)*cos(q_3)*sin(q_2)))*(1.0*cos(q_1)*cos(q_2)*sin(q_3) + 1.0*cos(q_1)*cos(q_3)*sin(q_2)) - 1.0*sin(q_1)*(0.0462*cos(q_1)^2 + 0.0462*sin(q_1)^2)) - 1.0*(1.0*cos(q_2)*sin(q_3) + 1.0*cos(q_3)*sin(q_2))*(0.0016*cos(q_1)*(1.0*cos(q_2)*sin(q_1)*sin(q_3) + 1.0*cos(q_3)*sin(q_1)*sin(q_2)) - 0.0016*sin(q_1)*(cos(q_1)*cos(q_2)*sin(q_3) + 1.0*cos(q_1)*cos(q_3)*sin(q_2))) + 1.0*(1.0*cos(q_2)*sin(q_3) + 1.0*cos(q_3)*sin(q_2))*(0.0016*cos(q_1)*(1.0*cos(q_2)*sin(q_1)*sin(q_3) + 1.0*cos(q_3)*sin(q_1)*sin(q_2)) - 0.0016*sin(q_1)*(1.0*cos(q_1)*cos(q_2)*sin(q_3) + cos(q_1)*cos(q_3)*sin(q_2))) + 1.0*cos(q_1)*(1.0*sin(q_1)*(0.0462*cos(q_1)^2 + 0.0462*sin(q_1)^2) - 1.0*(0.0462*cos(q_1)*(1.0*cos(q_2)*sin(q_1)*sin(q_3) + 1.0*cos(q_3)*sin(q_1)*sin(q_2)) - 0.0462*sin(q_1)*(1.0*cos(q_1)*cos(q_2)*sin(q_3) + 1.0*cos(q_1)*cos(q_3)*sin(q_2)))*(1.0*cos(q_1)*cos(q_2)*sin(q_3) + 1.0*cos(q_1)*cos(q_3)*sin(q_2)) + (cos(q_1)*cos(q_2)*cos(q_3) - 1.0*cos(q_1)*sin(q_2)*sin(q_3))*(0.0016*cos(q_1)*(1.0*sin(q_1)*sin(q_2)*sin(q_3) - 1.0*cos(q_2)*cos(q_3)*sin(q_1)) + 0.0016*sin(q_1)*(cos(q_1)*cos(q_2)*cos(q_3) - 1.0*cos(q_1)*sin(q_2)*sin(q_3))))), 0.5*dq_1*(1.0*sin(q_1)*((1.0*sin(q_1)*sin(q_2)*sin(q_3) - 1.0*cos(q_2)*cos(q_3)*sin(q_1))*(0.0016*cos(q_1)*(1.0*sin(q_1)*sin(q_2)*sin(q_3) - 1.0*cos(q_2)*cos(q_3)*sin(q_1)) + 0.0016*sin(q_1)*(cos(q_1)*cos(q_2)*cos(q_3) - 1.0*cos(q_1)*sin(q_2)*sin(q_3))) + 1.0*(0.0462*cos(q_1)*(1.0*cos(q_2)*sin(q_1)*sin(q_3) + 1.0*cos(q_3)*sin(q_1)*sin(q_2)) - 0.0462*sin(q_1)*(1.0*cos(q_1)*cos(q_2)*sin(q_3) + 1.0*cos(q_1)*cos(q_3)*sin(q_2)))*(1.0*cos(q_2)*sin(q_1)*sin(q_3) + 1.0*cos(q_3)*sin(q_1)*sin(q_2)) + 1.0*cos(q_1)*(0.0462*cos(q_1)^2 + 0.0462*sin(q_1)^2) + 1.0*(cos(q_1)*cos(q_2)*cos(q_3) - 1.0*cos(q_1)*sin(q_2)*sin(q_3))*(0.0016*cos(q_1)*(cos(q_1)*cos(q_2)*cos(q_3) - 1.0*cos(q_1)*sin(q_2)*sin(q_3)) - 0.0016*cos(q_1)*(1.0*cos(q_1)*cos(q_2)*cos(q_3) - 1.0*cos(q_1)*sin(q_2)*sin(q_3)))) - 1.0*sin(q_1)*((1.0*sin(q_1)*sin(q_2)*sin(q_3) - 1.0*cos(q_2)*cos(q_3)*sin(q_1))*(0.0016*cos(q_1)*(1.0*sin(q_1)*sin(q_2)*sin(q_3) - 1.0*cos(q_2)*cos(q_3)*sin(q_1)) + 0.0016*sin(q_1)*(cos(q_1)*cos(q_2)*cos(q_3) - 1.0*cos(q_1)*sin(q_2)*sin(q_3))) + (0.0462*cos(q_1)*(1.0*cos(q_2)*sin(q_1)*sin(q_3) + 1.0*cos(q_3)*sin(q_1)*sin(q_2)) - 0.0462*sin(q_1)*(1.0*cos(q_1)*cos(q_2)*sin(q_3) + 1.0*cos(q_1)*cos(q_3)*sin(q_2)))*(1.0*cos(q_2)*sin(q_1)*sin(q_3) + 1.0*cos(q_3)*sin(q_1)*sin(q_2)) + 1.0*cos(q_1)*(0.0462*cos(q_1)^2 + 0.0462*sin(q_1)^2)) + 1.0*cos(q_1)*((0.0016*cos(q_1)*(cos(q_1)*cos(q_2)*cos(q_3) - 1.0*cos(q_1)*sin(q_2)*sin(q_3)) - 0.0016*cos(q_1)*(1.0*cos(q_1)*cos(q_2)*cos(q_3) - 1.0*cos(q_1)*sin(q_2)*sin(q_3)))*(1.0*sin(q_1)*sin(q_2)*sin(q_3) - 1.0*cos(q_2)*cos(q_3)*sin(q_1)) - 1.0*(1.0*cos(q_1)*cos(q_2)*cos(q_3) - 1.0*cos(q_1)*sin(q_2)*sin(q_3))*(0.0016*cos(q_1)*(1.0*sin(q_1)*sin(q_2)*sin(q_3) - 1.0*cos(q_2)*cos(q_3)*sin(q_1)) + 0.0016*sin(q_1)*(cos(q_1)*cos(q_2)*cos(q_3) - 1.0*cos(q_1)*sin(q_2)*sin(q_3))) + 1.0*(0.0462*cos(q_1)*(1.0*cos(q_2)*sin(q_1)*sin(q_3) + 1.0*cos(q_3)*sin(q_1)*sin(q_2)) - 0.0462*sin(q_1)*(1.0*cos(q_1)*cos(q_2)*sin(q_3) + 1.0*cos(q_1)*cos(q_3)*sin(q_2)))*(1.0*cos(q_1)*cos(q_2)*sin(q_3) + 1.0*cos(q_1)*cos(q_3)*sin(q_2)) - 1.0*sin(q_1)*(0.0462*cos(q_1)^2 + 0.0462*sin(q_1)^2)) + 1.0*cos(q_1)*((0.0462*cos(q_2)*cos(q_3) - 0.0462*sin(q_2)*sin(q_3))*(1.0*sin(q_1)*sin(q_2)*sin(q_3) - 1.0*cos(q_2)*cos(q_3)*sin(q_1)) + (0.0462*cos(q_2)*sin(q_3) + 0.0462*cos(q_3)*sin(q_2))*(1.0*cos(q_2)*sin(q_1)*sin(q_3) + 1.0*cos(q_3)*sin(q_1)*sin(q_2)) - 1.0*(0.0016*cos(q_2)*cos(q_3) - 0.0016*sin(q_2)*sin(q_3))*(1.0*sin(q_1)*sin(q_2)*sin(q_3) - 1.0*cos(q_2)*cos(q_3)*sin(q_1)) - 1.0*(0.0016*cos(q_2)*sin(q_3) + 0.0016*cos(q_3)*sin(q_2))*(1.0*cos(q_2)*sin(q_1)*sin(q_3) + 1.0*cos(q_3)*sin(q_1)*sin(q_2))) + 1.0*(1.0*cos(q_2)*cos(q_3) - 1.0*sin(q_2)*sin(q_3))*(0.0016*cos(q_1)*(1.0*sin(q_1)*sin(q_2)*sin(q_3) - 1.0*cos(q_2)*cos(q_3)*sin(q_1)) + 0.0016*sin(q_1)*(cos(q_1)*cos(q_2)*cos(q_3) - 1.0*cos(q_1)*sin(q_2)*sin(q_3))) + 1.0*(1.0*cos(q_2)*sin(q_3) + 1.0*cos(q_3)*sin(q_2))*(0.0016*cos(q_1)*(1.0*cos(q_2)*sin(q_1)*sin(q_3) + 1.0*cos(q_3)*sin(q_1)*sin(q_2)) - 0.0016*sin(q_1)*(1.0*cos(q_1)*cos(q_2)*sin(q_3) + cos(q_1)*cos(q_3)*sin(q_2))) - 1.0*(1.0*cos(q_2)*cos(q_3) - 1.0*sin(q_2)*sin(q_3))*(0.0462*cos(q_1)*(1.0*sin(q_1)*sin(q_2)*sin(q_3) - 1.0*cos(q_2)*cos(q_3)*sin(q_1)) + 0.0462*sin(q_1)*(1.0*cos(q_1)*cos(q_2)*cos(q_3) - 1.0*cos(q_1)*sin(q_2)*sin(q_3))) - 1.0*(1.0*cos(q_2)*sin(q_3) + 1.0*cos(q_3)*sin(q_2))*(0.0462*cos(q_1)*(1.0*cos(q_2)*sin(q_1)*sin(q_3) + 1.0*cos(q_3)*sin(q_1)*sin(q_2)) - 0.0462*sin(q_1)*(1.0*cos(q_1)*cos(q_2)*sin(q_3) + 1.0*cos(q_1)*cos(q_3)*sin(q_2))) - 1.0*sin(q_1)*((0.0016*cos(q_2)*cos(q_3) - 0.0016*sin(q_2)*sin(q_3))*(cos(q_1)*cos(q_2)*cos(q_3) - 1.0*cos(q_1)*sin(q_2)*sin(q_3)) - 1.0*(0.0016*cos(q_2)*sin(q_3) + 0.0016*cos(q_3)*sin(q_2))*(cos(q_1)*cos(q_2)*sin(q_3) + 1.0*cos(q_1)*cos(q_3)*sin(q_2)) - 1.0*(0.0462*cos(q_2)*cos(q_3) - 0.0462*sin(q_2)*sin(q_3))*(1.0*cos(q_1)*cos(q_2)*cos(q_3) - 1.0*cos(q_1)*sin(q_2)*sin(q_3)) + 1.0*(0.0462*cos(q_2)*sin(q_3) + 0.0462*cos(q_3)*sin(q_2))*(1.0*cos(q_1)*cos(q_2)*sin(q_3) + 1.0*cos(q_1)*cos(q_3)*sin(q_2))) + 1.0*cos(q_1)*(1.0*sin(q_1)*(0.0462*cos(q_1)^2 + 0.0462*sin(q_1)^2) - 1.0*(0.0462*cos(q_1)*(1.0*cos(q_2)*sin(q_1)*sin(q_3) + 1.0*cos(q_3)*sin(q_1)*sin(q_2)) - 0.0462*sin(q_1)*(1.0*cos(q_1)*cos(q_2)*sin(q_3) + 1.0*cos(q_1)*cos(q_3)*sin(q_2)))*(1.0*cos(q_1)*cos(q_2)*sin(q_3) + 1.0*cos(q_1)*cos(q_3)*sin(q_2)) + (cos(q_1)*cos(q_2)*cos(q_3) - 1.0*cos(q_1)*sin(q_2)*sin(q_3))*(0.0016*cos(q_1)*(1.0*sin(q_1)*sin(q_2)*sin(q_3) - 1.0*cos(q_2)*cos(q_3)*sin(q_1)) + 0.0016*sin(q_1)*(cos(q_1)*cos(q_2)*cos(q_3) - 1.0*cos(q_1)*sin(q_2)*sin(q_3)))) - 2.275*cos(q_1)*(0.0265*cos(q_1) + 1.0*sin(q_1)*(0.2723*sin(q_2)*sin(q_3) - 1.0*cos(q_2)*(0.2723*cos(q_3) + 0.425)))*(0.2723*cos(q_2)*cos(q_3) - 0.2723*sin(q_2)*sin(q_3)) - 2.275*sin(q_1)*(0.0265*sin(q_1) - 1.0*cos(q_1)*(0.2723*sin(q_2)*sin(q_3) - 1.0*cos(q_2)*(0.2723*cos(q_3) + 0.425)))*(0.2723*cos(q_2)*cos(q_3) - 0.2723*sin(q_2)*sin(q_3)) + 1.0*cos(q_1)*(0.2723*cos(q_2)*cos(q_3) - 0.2723*sin(q_2)*sin(q_3))*(0.06029*cos(q_1) + 2.275*sin(q_1)*(0.2723*sin(q_2)*sin(q_3) - 1.0*cos(q_2)*(0.2723*cos(q_3) + 0.425))) + 1.0*sin(q_1)*(0.2723*cos(q_2)*cos(q_3) - 0.2723*sin(q_2)*sin(q_3))*(0.06029*sin(q_1) - 2.275*cos(q_1)*(0.2723*sin(q_2)*sin(q_3) - 1.0*cos(q_2)*(0.2723*cos(q_3) + 0.425)))) - 0.5*dq_2*((0.2723*cos(q_2)*sin(q_3) + 0.2723*cos(q_3)*sin(q_2))*(0.6195*sin(q_2)*sin(q_3) - 2.275*cos(q_2)*(0.2723*cos(q_3) + 0.425)) + 2.0*(0.6195*cos(q_2)*cos(q_3) - 0.6195*sin(q_2)*sin(q_3))*(0.2723*cos(q_2)*sin(q_3) + 1.0*sin(q_2)*(0.2723*cos(q_3) + 0.425)) - 2.0*(0.6195*cos(q_2)*sin(q_3) + 0.6195*cos(q_3)*sin(q_2))*(0.2723*sin(q_2)*sin(q_3) - 1.0*cos(q_2)*(0.2723*cos(q_3) + 0.425)) + (0.6195*cos(q_2)*sin(q_3) + 0.6195*cos(q_3)*sin(q_2))*(0.2723*sin(q_2)*sin(q_3) - 1.0*cos(q_2)*(0.2723*cos(q_3) + 0.425)) + 1.0*cos(q_1)*((1.0*cos(q_2)*sin(q_1)*sin(q_3) + 1.0*cos(q_3)*sin(q_1)*sin(q_2))*(0.0016*cos(q_1)*(1.0*sin(q_1)*sin(q_2)*sin(q_3) - 1.0*cos(q_2)*cos(q_3)*sin(q_1)) + 0.0016*sin(q_1)*(cos(q_1)*cos(q_2)*cos(q_3) - 1.0*cos(q_1)*sin(q_2)*sin(q_3))) + (1.0*sin(q_1)*sin(q_2)*sin(q_3) - 1.0*cos(q_2)*cos(q_3)*sin(q_1))*(0.0016*cos(q_1)*(1.0*cos(q_2)*sin(q_1)*sin(q_3) + 1.0*cos(q_3)*sin(q_1)*sin(q_2)) - 0.0016*sin(q_1)*(cos(q_1)*cos(q_2)*sin(q_3) + 1.0*cos(q_1)*cos(q_3)*sin(q_2))) - 1.0*(0.0462*cos(q_1)*(1.0*cos(q_2)*sin(q_1)*sin(q_3) + 1.0*cos(q_3)*sin(q_1)*sin(q_2)) - 0.0462*sin(q_1)*(1.0*cos(q_1)*cos(q_2)*sin(q_3) + 1.0*cos(q_1)*cos(q_3)*sin(q_2)))*(1.0*sin(q_1)*sin(q_2)*sin(q_3) - 1.0*cos(q_2)*cos(q_3)*sin(q_1)) - 1.0*(0.0462*cos(q_1)*(1.0*sin(q_1)*sin(q_2)*sin(q_3) - 1.0*cos(q_2)*cos(q_3)*sin(q_1)) + 0.0462*sin(q_1)*(1.0*cos(q_1)*cos(q_2)*cos(q_3) - 1.0*cos(q_1)*sin(q_2)*sin(q_3)))*(1.0*cos(q_2)*sin(q_1)*sin(q_3) + 1.0*cos(q_3)*sin(q_1)*sin(q_2))) - 2.0*cos(q_1)*((1.0*cos(q_2)*sin(q_1)*sin(q_3) + 1.0*cos(q_3)*sin(q_1)*sin(q_2))*(0.0016*cos(q_1)*(1.0*sin(q_1)*sin(q_2)*sin(q_3) - 1.0*cos(q_2)*cos(q_3)*sin(q_1)) + 0.0016*sin(q_1)*(cos(q_1)*cos(q_2)*cos(q_3) - 1.0*cos(q_1)*sin(q_2)*sin(q_3))) + (1.0*sin(q_1)*sin(q_2)*sin(q_3) - 1.0*cos(q_2)*cos(q_3)*sin(q_1))*(0.0016*cos(q_1)*(1.0*cos(q_2)*sin(q_1)*sin(q_3) + 1.0*cos(q_3)*sin(q_1)*sin(q_2)) - 0.0016*sin(q_1)*(1.0*cos(q_1)*cos(q_2)*sin(q_3) + cos(q_1)*cos(q_3)*sin(q_2))) - 1.0*(0.0462*cos(q_1)*(1.0*cos(q_2)*sin(q_1)*sin(q_3) + 1.0*cos(q_3)*sin(q_1)*sin(q_2)) - 0.0462*sin(q_1)*(1.0*cos(q_1)*cos(q_2)*sin(q_3) + 1.0*cos(q_1)*cos(q_3)*sin(q_2)))*(1.0*sin(q_1)*sin(q_2)*sin(q_3) - 1.0*cos(q_2)*cos(q_3)*sin(q_1)) - 1.0*(0.0462*cos(q_1)*(1.0*sin(q_1)*sin(q_2)*sin(q_3) - 1.0*cos(q_2)*cos(q_3)*sin(q_1)) + 0.0462*sin(q_1)*(1.0*cos(q_1)*cos(q_2)*cos(q_3) - 1.0*cos(q_1)*sin(q_2)*sin(q_3)))*(1.0*cos(q_2)*sin(q_1)*sin(q_3) + 1.0*cos(q_3)*sin(q_1)*sin(q_2))) - 1.0*sin(q_1)*(1.0*(0.0462*cos(q_1)*(1.0*cos(q_2)*sin(q_1)*sin(q_3) + 1.0*cos(q_3)*sin(q_1)*sin(q_2)) - 0.0462*sin(q_1)*(1.0*cos(q_1)*cos(q_2)*sin(q_3) + 1.0*cos(q_1)*cos(q_3)*sin(q_2)))*(1.0*cos(q_1)*cos(q_2)*cos(q_3) - 1.0*cos(q_1)*sin(q_2)*sin(q_3)) - 1.0*(0.0462*cos(q_1)*(1.0*sin(q_1)*sin(q_2)*sin(q_3) - 1.0*cos(q_2)*cos(q_3)*sin(q_1)) + 0.0462*sin(q_1)*(1.0*cos(q_1)*cos(q_2)*cos(q_3) - 1.0*cos(q_1)*sin(q_2)*sin(q_3)))*(1.0*cos(q_1)*cos(q_2)*sin(q_3) + 1.0*cos(q_1)*cos(q_3)*sin(q_2)) - 1.0*(cos(q_1)*cos(q_2)*cos(q_3) - 1.0*cos(q_1)*sin(q_2)*sin(q_3))*(0.0016*cos(q_1)*(1.0*cos(q_2)*sin(q_1)*sin(q_3) + 1.0*cos(q_3)*sin(q_1)*sin(q_2)) - 0.0016*sin(q_1)*(cos(q_1)*cos(q_2)*sin(q_3) + 1.0*cos(q_1)*cos(q_3)*sin(q_2))) + (cos(q_1)*cos(q_2)*sin(q_3) + 1.0*cos(q_1)*cos(q_3)*sin(q_2))*(0.0016*cos(q_1)*(1.0*sin(q_1)*sin(q_2)*sin(q_3) - 1.0*cos(q_2)*cos(q_3)*sin(q_1)) + 0.0016*sin(q_1)*(cos(q_1)*cos(q_2)*cos(q_3) - 1.0*cos(q_1)*sin(q_2)*sin(q_3)))) + 2.0*sin(q_1)*(1.0*(0.0462*cos(q_1)*(1.0*cos(q_2)*sin(q_1)*sin(q_3) + 1.0*cos(q_3)*sin(q_1)*sin(q_2)) - 0.0462*sin(q_1)*(1.0*cos(q_1)*cos(q_2)*sin(q_3) + 1.0*cos(q_1)*cos(q_3)*sin(q_2)))*(1.0*cos(q_1)*cos(q_2)*cos(q_3) - 1.0*cos(q_1)*sin(q_2)*sin(q_3)) - 1.0*(0.0462*cos(q_1)*(1.0*sin(q_1)*sin(q_2)*sin(q_3) - 1.0*cos(q_2)*cos(q_3)*sin(q_1)) + 0.0462*sin(q_1)*(1.0*cos(q_1)*cos(q_2)*cos(q_3) - 1.0*cos(q_1)*sin(q_2)*sin(q_3)))*(1.0*cos(q_1)*cos(q_2)*sin(q_3) + 1.0*cos(q_1)*cos(q_3)*sin(q_2)) - 1.0*(cos(q_1)*cos(q_2)*cos(q_3) - 1.0*cos(q_1)*sin(q_2)*sin(q_3))*(0.0016*cos(q_1)*(1.0*cos(q_2)*sin(q_1)*sin(q_3) + 1.0*cos(q_3)*sin(q_1)*sin(q_2)) - 0.0016*sin(q_1)*(1.0*cos(q_1)*cos(q_2)*sin(q_3) + cos(q_1)*cos(q_3)*sin(q_2))) + (1.0*cos(q_1)*cos(q_2)*sin(q_3) + cos(q_1)*cos(q_3)*sin(q_2))*(0.0016*cos(q_1)*(1.0*sin(q_1)*sin(q_2)*sin(q_3) - 1.0*cos(q_2)*cos(q_3)*sin(q_1)) + 0.0016*sin(q_1)*(cos(q_1)*cos(q_2)*cos(q_3) - 1.0*cos(q_1)*sin(q_2)*sin(q_3)))) + 4.55*cos(q_1)^2*(0.2723*cos(q_2)*sin(q_3) + 0.2723*cos(q_3)*sin(q_2))*(0.2723*sin(q_2)*sin(q_3) - 1.0*cos(q_2)*(0.2723*cos(q_3) + 0.425)) + 4.55*sin(q_1)^2*(0.2723*cos(q_2)*sin(q_3) + 0.2723*cos(q_3)*sin(q_2))*(0.2723*sin(q_2)*sin(q_3) - 1.0*cos(q_2)*(0.2723*cos(q_3) + 0.425))) + 0.5*dq_3*(1.0*cos(q_1)*((1.0*cos(q_2)*sin(q_1)*sin(q_3) + 1.0*cos(q_3)*sin(q_1)*sin(q_2))*(0.0016*cos(q_1)*(1.0*sin(q_1)*sin(q_2)*sin(q_3) - 1.0*cos(q_2)*cos(q_3)*sin(q_1)) + 0.0016*sin(q_1)*(cos(q_1)*cos(q_2)*cos(q_3) - 1.0*cos(q_1)*sin(q_2)*sin(q_3))) + (1.0*sin(q_1)*sin(q_2)*sin(q_3) - 1.0*cos(q_2)*cos(q_3)*sin(q_1))*(0.0016*cos(q_1)*(1.0*cos(q_2)*sin(q_1)*sin(q_3) + 1.0*cos(q_3)*sin(q_1)*sin(q_2)) - 0.0016*sin(q_1)*(1.0*cos(q_1)*cos(q_2)*sin(q_3) + cos(q_1)*cos(q_3)*sin(q_2))) - 1.0*(0.0462*cos(q_1)*(1.0*cos(q_2)*sin(q_1)*sin(q_3) + 1.0*cos(q_3)*sin(q_1)*sin(q_2)) - 0.0462*sin(q_1)*(1.0*cos(q_1)*cos(q_2)*sin(q_3) + 1.0*cos(q_1)*cos(q_3)*sin(q_2)))*(1.0*sin(q_1)*sin(q_2)*sin(q_3) - 1.0*cos(q_2)*cos(q_3)*sin(q_1)) - 1.0*(0.0462*cos(q_1)*(1.0*sin(q_1)*sin(q_2)*sin(q_3) - 1.0*cos(q_2)*cos(q_3)*sin(q_1)) + 0.0462*sin(q_1)*(1.0*cos(q_1)*cos(q_2)*cos(q_3) - 1.0*cos(q_1)*sin(q_2)*sin(q_3)))*(1.0*cos(q_2)*sin(q_1)*sin(q_3) + 1.0*cos(q_3)*sin(q_1)*sin(q_2))) - 1.0*sin(q_1)*(1.0*(0.0462*cos(q_1)*(1.0*cos(q_2)*sin(q_1)*sin(q_3) + 1.0*cos(q_3)*sin(q_1)*sin(q_2)) - 0.0462*sin(q_1)*(1.0*cos(q_1)*cos(q_2)*sin(q_3) + 1.0*cos(q_1)*cos(q_3)*sin(q_2)))*(1.0*cos(q_1)*cos(q_2)*cos(q_3) - 1.0*cos(q_1)*sin(q_2)*sin(q_3)) - 1.0*(0.0462*cos(q_1)*(1.0*sin(q_1)*sin(q_2)*sin(q_3) - 1.0*cos(q_2)*cos(q_3)*sin(q_1)) + 0.0462*sin(q_1)*(1.0*cos(q_1)*cos(q_2)*cos(q_3) - 1.0*cos(q_1)*sin(q_2)*sin(q_3)))*(1.0*cos(q_1)*cos(q_2)*sin(q_3) + 1.0*cos(q_1)*cos(q_3)*sin(q_2)) - 1.0*(cos(q_1)*cos(q_2)*cos(q_3) - 1.0*cos(q_1)*sin(q_2)*sin(q_3))*(0.0016*cos(q_1)*(1.0*cos(q_2)*sin(q_1)*sin(q_3) + 1.0*cos(q_3)*sin(q_1)*sin(q_2)) - 0.0016*sin(q_1)*(1.0*cos(q_1)*cos(q_2)*sin(q_3) + cos(q_1)*cos(q_3)*sin(q_2))) + (1.0*cos(q_1)*cos(q_2)*sin(q_3) + cos(q_1)*cos(q_3)*sin(q_2))*(0.0016*cos(q_1)*(1.0*sin(q_1)*sin(q_2)*sin(q_3) - 1.0*cos(q_2)*cos(q_3)*sin(q_1)) + 0.0016*sin(q_1)*(cos(q_1)*cos(q_2)*cos(q_3) - 1.0*cos(q_1)*sin(q_2)*sin(q_3)))) - 1.0*(0.2723*cos(q_2)*cos(q_3) - 0.2723*sin(q_2)*sin(q_3))*(0.6195*cos(q_2)*sin(q_3) + 0.6195*cos(q_3)*sin(q_2)) - 1.0*(0.2723*cos(q_2)*sin(q_3) + 0.2723*cos(q_3)*sin(q_2))*(0.6195*cos(q_2)*cos(q_3) - 0.6195*sin(q_2)*sin(q_3)) + 4.55*cos(q_1)^2*(0.2723*cos(q_2)*cos(q_3) - 0.2723*sin(q_2)*sin(q_3))*(0.2723*cos(q_2)*sin(q_3) + 0.2723*cos(q_3)*sin(q_2)) + 4.55*sin(q_1)^2*(0.2723*cos(q_2)*cos(q_3) - 0.2723*sin(q_2)*sin(q_3))*(0.2723*cos(q_2)*sin(q_3) + 0.2723*cos(q_3)*sin(q_2))),                                                                                                                                                                                                                                                                                                                                                                                                                                                                                                                                                                                                                                                                                                                                                                                                                                                                                                                                                                                                                                                                                                                                                                                                                                                                                                                                                                                                                                                                                                                                                                                                                                                                                                                                                                                                                                                                                                                                     0.5*dq_1*(1.0*sin(q_1)*((1.0*sin(q_1)*sin(q_2)*sin(q_3) - 1.0*cos(q_2)*cos(q_3)*sin(q_1))*(0.0016*cos(q_1)*(1.0*sin(q_1)*sin(q_2)*sin(q_3) - 1.0*cos(q_2)*cos(q_3)*sin(q_1)) + 0.0016*sin(q_1)*(cos(q_1)*cos(q_2)*cos(q_3) - 1.0*cos(q_1)*sin(q_2)*sin(q_3))) + 1.0*(0.0462*cos(q_1)*(1.0*cos(q_2)*sin(q_1)*sin(q_3) + 1.0*cos(q_3)*sin(q_1)*sin(q_2)) - 0.0462*sin(q_1)*(1.0*cos(q_1)*cos(q_2)*sin(q_3) + 1.0*cos(q_1)*cos(q_3)*sin(q_2)))*(1.0*cos(q_2)*sin(q_1)*sin(q_3) + 1.0*cos(q_3)*sin(q_1)*sin(q_2)) + 1.0*cos(q_1)*(0.0462*cos(q_1)^2 + 0.0462*sin(q_1)^2) + 1.0*(cos(q_1)*cos(q_2)*cos(q_3) - 1.0*cos(q_1)*sin(q_2)*sin(q_3))*(0.0016*cos(q_1)*(cos(q_1)*cos(q_2)*cos(q_3) - 1.0*cos(q_1)*sin(q_2)*sin(q_3)) - 0.0016*cos(q_1)*(1.0*cos(q_1)*cos(q_2)*cos(q_3) - 1.0*cos(q_1)*sin(q_2)*sin(q_3)))) - 1.0*sin(q_1)*((1.0*sin(q_1)*sin(q_2)*sin(q_3) - 1.0*cos(q_2)*cos(q_3)*sin(q_1))*(0.0016*cos(q_1)*(1.0*sin(q_1)*sin(q_2)*sin(q_3) - 1.0*cos(q_2)*cos(q_3)*sin(q_1)) + 0.0016*sin(q_1)*(cos(q_1)*cos(q_2)*cos(q_3) - 1.0*cos(q_1)*sin(q_2)*sin(q_3))) + (0.0462*cos(q_1)*(1.0*cos(q_2)*sin(q_1)*sin(q_3) + 1.0*cos(q_3)*sin(q_1)*sin(q_2)) - 0.0462*sin(q_1)*(1.0*cos(q_1)*cos(q_2)*sin(q_3) + 1.0*cos(q_1)*cos(q_3)*sin(q_2)))*(1.0*cos(q_2)*sin(q_1)*sin(q_3) + 1.0*cos(q_3)*sin(q_1)*sin(q_2)) + 1.0*cos(q_1)*(0.0462*cos(q_1)^2 + 0.0462*sin(q_1)^2)) + 1.0*cos(q_1)*((0.0016*cos(q_1)*(cos(q_1)*cos(q_2)*cos(q_3) - 1.0*cos(q_1)*sin(q_2)*sin(q_3)) - 0.0016*cos(q_1)*(1.0*cos(q_1)*cos(q_2)*cos(q_3) - 1.0*cos(q_1)*sin(q_2)*sin(q_3)))*(1.0*sin(q_1)*sin(q_2)*sin(q_3) - 1.0*cos(q_2)*cos(q_3)*sin(q_1)) - 1.0*(1.0*cos(q_1)*cos(q_2)*cos(q_3) - 1.0*cos(q_1)*sin(q_2)*sin(q_3))*(0.0016*cos(q_1)*(1.0*sin(q_1)*sin(q_2)*sin(q_3) - 1.0*cos(q_2)*cos(q_3)*sin(q_1)) + 0.0016*sin(q_1)*(cos(q_1)*cos(q_2)*cos(q_3) - 1.0*cos(q_1)*sin(q_2)*sin(q_3))) + 1.0*(0.0462*cos(q_1)*(1.0*cos(q_2)*sin(q_1)*sin(q_3) + 1.0*cos(q_3)*sin(q_1)*sin(q_2)) - 0.0462*sin(q_1)*(1.0*cos(q_1)*cos(q_2)*sin(q_3) + 1.0*cos(q_1)*cos(q_3)*sin(q_2)))*(1.0*cos(q_1)*cos(q_2)*sin(q_3) + 1.0*cos(q_1)*cos(q_3)*sin(q_2)) - 1.0*sin(q_1)*(0.0462*cos(q_1)^2 + 0.0462*sin(q_1)^2)) + 1.0*cos(q_1)*((0.0462*cos(q_2)*cos(q_3) - 0.0462*sin(q_2)*sin(q_3))*(1.0*sin(q_1)*sin(q_2)*sin(q_3) - 1.0*cos(q_2)*cos(q_3)*sin(q_1)) + (0.0462*cos(q_2)*sin(q_3) + 0.0462*cos(q_3)*sin(q_2))*(1.0*cos(q_2)*sin(q_1)*sin(q_3) + 1.0*cos(q_3)*sin(q_1)*sin(q_2)) - 1.0*(0.0016*cos(q_2)*cos(q_3) - 0.0016*sin(q_2)*sin(q_3))*(1.0*sin(q_1)*sin(q_2)*sin(q_3) - 1.0*cos(q_2)*cos(q_3)*sin(q_1)) - 1.0*(0.0016*cos(q_2)*sin(q_3) + 0.0016*cos(q_3)*sin(q_2))*(1.0*cos(q_2)*sin(q_1)*sin(q_3) + 1.0*cos(q_3)*sin(q_1)*sin(q_2))) + 1.0*(1.0*cos(q_2)*cos(q_3) - 1.0*sin(q_2)*sin(q_3))*(0.0016*cos(q_1)*(1.0*sin(q_1)*sin(q_2)*sin(q_3) - 1.0*cos(q_2)*cos(q_3)*sin(q_1)) + 0.0016*sin(q_1)*(cos(q_1)*cos(q_2)*cos(q_3) - 1.0*cos(q_1)*sin(q_2)*sin(q_3))) + 1.0*(1.0*cos(q_2)*sin(q_3) + 1.0*cos(q_3)*sin(q_2))*(0.0016*cos(q_1)*(1.0*cos(q_2)*sin(q_1)*sin(q_3) + 1.0*cos(q_3)*sin(q_1)*sin(q_2)) - 0.0016*sin(q_1)*(cos(q_1)*cos(q_2)*sin(q_3) + 1.0*cos(q_1)*cos(q_3)*sin(q_2))) - 1.0*(1.0*cos(q_2)*cos(q_3) - 1.0*sin(q_2)*sin(q_3))*(0.0462*cos(q_1)*(1.0*sin(q_1)*sin(q_2)*sin(q_3) - 1.0*cos(q_2)*cos(q_3)*sin(q_1)) + 0.0462*sin(q_1)*(1.0*cos(q_1)*cos(q_2)*cos(q_3) - 1.0*cos(q_1)*sin(q_2)*sin(q_3))) - 1.0*(1.0*cos(q_2)*sin(q_3) + 1.0*cos(q_3)*sin(q_2))*(0.0462*cos(q_1)*(1.0*cos(q_2)*sin(q_1)*sin(q_3) + 1.0*cos(q_3)*sin(q_1)*sin(q_2)) - 0.0462*sin(q_1)*(1.0*cos(q_1)*cos(q_2)*sin(q_3) + 1.0*cos(q_1)*cos(q_3)*sin(q_2))) - 1.0*sin(q_1)*((0.0016*cos(q_2)*cos(q_3) - 0.0016*sin(q_2)*sin(q_3))*(cos(q_1)*cos(q_2)*cos(q_3) - 1.0*cos(q_1)*sin(q_2)*sin(q_3)) - 1.0*(0.0016*cos(q_2)*sin(q_3) + 0.0016*cos(q_3)*sin(q_2))*(cos(q_1)*cos(q_2)*sin(q_3) + 1.0*cos(q_1)*cos(q_3)*sin(q_2)) - 1.0*(0.0462*cos(q_2)*cos(q_3) - 0.0462*sin(q_2)*sin(q_3))*(1.0*cos(q_1)*cos(q_2)*cos(q_3) - 1.0*cos(q_1)*sin(q_2)*sin(q_3)) + 1.0*(0.0462*cos(q_2)*sin(q_3) + 0.0462*cos(q_3)*sin(q_2))*(1.0*cos(q_1)*cos(q_2)*sin(q_3) + 1.0*cos(q_1)*cos(q_3)*sin(q_2))) + 1.0*cos(q_1)*(1.0*sin(q_1)*(0.0462*cos(q_1)^2 + 0.0462*sin(q_1)^2) - 1.0*(0.0462*cos(q_1)*(1.0*cos(q_2)*sin(q_1)*sin(q_3) + 1.0*cos(q_3)*sin(q_1)*sin(q_2)) - 0.0462*sin(q_1)*(1.0*cos(q_1)*cos(q_2)*sin(q_3) + 1.0*cos(q_1)*cos(q_3)*sin(q_2)))*(1.0*cos(q_1)*cos(q_2)*sin(q_3) + 1.0*cos(q_1)*cos(q_3)*sin(q_2)) + (cos(q_1)*cos(q_2)*cos(q_3) - 1.0*cos(q_1)*sin(q_2)*sin(q_3))*(0.0016*cos(q_1)*(1.0*sin(q_1)*sin(q_2)*sin(q_3) - 1.0*cos(q_2)*cos(q_3)*sin(q_1)) + 0.0016*sin(q_1)*(cos(q_1)*cos(q_2)*cos(q_3) - 1.0*cos(q_1)*sin(q_2)*sin(q_3)))) - 2.275*cos(q_1)*(0.0265*cos(q_1) + 1.0*sin(q_1)*(0.2723*sin(q_2)*sin(q_3) - 1.0*cos(q_2)*(0.2723*cos(q_3) + 0.425)))*(0.2723*cos(q_2)*cos(q_3) - 0.2723*sin(q_2)*sin(q_3)) - 2.275*sin(q_1)*(0.0265*sin(q_1) - 1.0*cos(q_1)*(0.2723*sin(q_2)*sin(q_3) - 1.0*cos(q_2)*(0.2723*cos(q_3) + 0.425)))*(0.2723*cos(q_2)*cos(q_3) - 0.2723*sin(q_2)*sin(q_3)) + 1.0*cos(q_1)*(0.2723*cos(q_2)*cos(q_3) - 0.2723*sin(q_2)*sin(q_3))*(0.06029*cos(q_1) + 2.275*sin(q_1)*(0.2723*sin(q_2)*sin(q_3) - 1.0*cos(q_2)*(0.2723*cos(q_3) + 0.425))) + 1.0*sin(q_1)*(0.2723*cos(q_2)*cos(q_3) - 0.2723*sin(q_2)*sin(q_3))*(0.06029*sin(q_1) - 2.275*cos(q_1)*(0.2723*sin(q_2)*sin(q_3) - 1.0*cos(q_2)*(0.2723*cos(q_3) + 0.425)))) + 0.5*dq_2*(1.0*(0.6195*cos(q_2)*sin(q_3) + 0.6195*cos(q_3)*sin(q_2))*(0.2723*sin(q_2)*sin(q_3) - 1.0*cos(q_2)*(0.2723*cos(q_3) + 0.425)) - 1.0*(0.2723*cos(q_2)*sin(q_3) + 0.2723*cos(q_3)*sin(q_2))*(0.6195*sin(q_2)*sin(q_3) - 2.275*cos(q_2)*(0.2723*cos(q_3) + 0.425)) + 1.0*cos(q_1)*((1.0*cos(q_2)*sin(q_1)*sin(q_3) + 1.0*cos(q_3)*sin(q_1)*sin(q_2))*(0.0016*cos(q_1)*(1.0*sin(q_1)*sin(q_2)*sin(q_3) - 1.0*cos(q_2)*cos(q_3)*sin(q_1)) + 0.0016*sin(q_1)*(cos(q_1)*cos(q_2)*cos(q_3) - 1.0*cos(q_1)*sin(q_2)*sin(q_3))) + (1.0*sin(q_1)*sin(q_2)*sin(q_3) - 1.0*cos(q_2)*cos(q_3)*sin(q_1))*(0.0016*cos(q_1)*(1.0*cos(q_2)*sin(q_1)*sin(q_3) + 1.0*cos(q_3)*sin(q_1)*sin(q_2)) - 0.0016*sin(q_1)*(1.0*cos(q_1)*cos(q_2)*sin(q_3) + cos(q_1)*cos(q_3)*sin(q_2))) - 1.0*(0.0462*cos(q_1)*(1.0*cos(q_2)*sin(q_1)*sin(q_3) + 1.0*cos(q_3)*sin(q_1)*sin(q_2)) - 0.0462*sin(q_1)*(1.0*cos(q_1)*cos(q_2)*sin(q_3) + 1.0*cos(q_1)*cos(q_3)*sin(q_2)))*(1.0*sin(q_1)*sin(q_2)*sin(q_3) - 1.0*cos(q_2)*cos(q_3)*sin(q_1)) - 1.0*(0.0462*cos(q_1)*(1.0*sin(q_1)*sin(q_2)*sin(q_3) - 1.0*cos(q_2)*cos(q_3)*sin(q_1)) + 0.0462*sin(q_1)*(1.0*cos(q_1)*cos(q_2)*cos(q_3) - 1.0*cos(q_1)*sin(q_2)*sin(q_3)))*(1.0*cos(q_2)*sin(q_1)*sin(q_3) + 1.0*cos(q_3)*sin(q_1)*sin(q_2))) - 1.0*sin(q_1)*(1.0*(0.0462*cos(q_1)*(1.0*cos(q_2)*sin(q_1)*sin(q_3) + 1.0*cos(q_3)*sin(q_1)*sin(q_2)) - 0.0462*sin(q_1)*(1.0*cos(q_1)*cos(q_2)*sin(q_3) + 1.0*cos(q_1)*cos(q_3)*sin(q_2)))*(1.0*cos(q_1)*cos(q_2)*cos(q_3) - 1.0*cos(q_1)*sin(q_2)*sin(q_3)) - 1.0*(0.0462*cos(q_1)*(1.0*sin(q_1)*sin(q_2)*sin(q_3) - 1.0*cos(q_2)*cos(q_3)*sin(q_1)) + 0.0462*sin(q_1)*(1.0*cos(q_1)*cos(q_2)*cos(q_3) - 1.0*cos(q_1)*sin(q_2)*sin(q_3)))*(1.0*cos(q_1)*cos(q_2)*sin(q_3) + 1.0*cos(q_1)*cos(q_3)*sin(q_2)) - 1.0*(cos(q_1)*cos(q_2)*cos(q_3) - 1.0*cos(q_1)*sin(q_2)*sin(q_3))*(0.0016*cos(q_1)*(1.0*cos(q_2)*sin(q_1)*sin(q_3) + 1.0*cos(q_3)*sin(q_1)*sin(q_2)) - 0.0016*sin(q_1)*(1.0*cos(q_1)*cos(q_2)*sin(q_3) + cos(q_1)*cos(q_3)*sin(q_2))) + (1.0*cos(q_1)*cos(q_2)*sin(q_3) + cos(q_1)*cos(q_3)*sin(q_2))*(0.0016*cos(q_1)*(1.0*sin(q_1)*sin(q_2)*sin(q_3) - 1.0*cos(q_2)*cos(q_3)*sin(q_1)) + 0.0016*sin(q_1)*(cos(q_1)*cos(q_2)*cos(q_3) - 1.0*cos(q_1)*sin(q_2)*sin(q_3)))) - 1.0*(0.2723*cos(q_2)*cos(q_3) - 0.2723*sin(q_2)*sin(q_3))*(0.6195*cos(q_2)*sin(q_3) + 0.6195*cos(q_3)*sin(q_2)) + 1.0*(0.2723*cos(q_2)*cos(q_3) - 0.2723*sin(q_2)*sin(q_3))*(0.6195*cos(q_2)*sin(q_3) + 0.6195*cos(q_3)*sin(q_2)) - 2.0*(0.2723*cos(q_2)*sin(q_3) + 0.2723*cos(q_3)*sin(q_2))*(0.6195*cos(q_2)*cos(q_3) - 0.6195*sin(q_2)*sin(q_3)) + 4.55*cos(q_1)^2*(0.2723*cos(q_2)*cos(q_3) - 0.2723*sin(q_2)*sin(q_3))*(0.2723*cos(q_2)*sin(q_3) + 0.2723*cos(q_3)*sin(q_2)) + 4.55*sin(q_1)^2*(0.2723*cos(q_2)*cos(q_3) - 0.2723*sin(q_2)*sin(q_3))*(0.2723*cos(q_2)*sin(q_3) + 0.2723*cos(q_3)*sin(q_2))) + 0.5*dq_3*(1.0*cos(q_1)*((1.0*cos(q_2)*sin(q_1)*sin(q_3) + 1.0*cos(q_3)*sin(q_1)*sin(q_2))*(0.0016*cos(q_1)*(1.0*sin(q_1)*sin(q_2)*sin(q_3) - 1.0*cos(q_2)*cos(q_3)*sin(q_1)) + 0.0016*sin(q_1)*(cos(q_1)*cos(q_2)*cos(q_3) - 1.0*cos(q_1)*sin(q_2)*sin(q_3))) + (1.0*sin(q_1)*sin(q_2)*sin(q_3) - 1.0*cos(q_2)*cos(q_3)*sin(q_1))*(0.0016*cos(q_1)*(1.0*cos(q_2)*sin(q_1)*sin(q_3) + 1.0*cos(q_3)*sin(q_1)*sin(q_2)) - 0.0016*sin(q_1)*(cos(q_1)*cos(q_2)*sin(q_3) + 1.0*cos(q_1)*cos(q_3)*sin(q_2))) - 1.0*(0.0462*cos(q_1)*(1.0*cos(q_2)*sin(q_1)*sin(q_3) + 1.0*cos(q_3)*sin(q_1)*sin(q_2)) - 0.0462*sin(q_1)*(1.0*cos(q_1)*cos(q_2)*sin(q_3) + 1.0*cos(q_1)*cos(q_3)*sin(q_2)))*(1.0*sin(q_1)*sin(q_2)*sin(q_3) - 1.0*cos(q_2)*cos(q_3)*sin(q_1)) - 1.0*(0.0462*cos(q_1)*(1.0*sin(q_1)*sin(q_2)*sin(q_3) - 1.0*cos(q_2)*cos(q_3)*sin(q_1)) + 0.0462*sin(q_1)*(1.0*cos(q_1)*cos(q_2)*cos(q_3) - 1.0*cos(q_1)*sin(q_2)*sin(q_3)))*(1.0*cos(q_2)*sin(q_1)*sin(q_3) + 1.0*cos(q_3)*sin(q_1)*sin(q_2))) - 1.0*sin(q_1)*(1.0*(0.0462*cos(q_1)*(1.0*cos(q_2)*sin(q_1)*sin(q_3) + 1.0*cos(q_3)*sin(q_1)*sin(q_2)) - 0.0462*sin(q_1)*(1.0*cos(q_1)*cos(q_2)*sin(q_3) + 1.0*cos(q_1)*cos(q_3)*sin(q_2)))*(1.0*cos(q_1)*cos(q_2)*cos(q_3) - 1.0*cos(q_1)*sin(q_2)*sin(q_3)) - 1.0*(0.0462*cos(q_1)*(1.0*sin(q_1)*sin(q_2)*sin(q_3) - 1.0*cos(q_2)*cos(q_3)*sin(q_1)) + 0.0462*sin(q_1)*(1.0*cos(q_1)*cos(q_2)*cos(q_3) - 1.0*cos(q_1)*sin(q_2)*sin(q_3)))*(1.0*cos(q_1)*cos(q_2)*sin(q_3) + 1.0*cos(q_1)*cos(q_3)*sin(q_2)) - 1.0*(cos(q_1)*cos(q_2)*cos(q_3) - 1.0*cos(q_1)*sin(q_2)*sin(q_3))*(0.0016*cos(q_1)*(1.0*cos(q_2)*sin(q_1)*sin(q_3) + 1.0*cos(q_3)*sin(q_1)*sin(q_2)) - 0.0016*sin(q_1)*(cos(q_1)*cos(q_2)*sin(q_3) + 1.0*cos(q_1)*cos(q_3)*sin(q_2))) + (cos(q_1)*cos(q_2)*sin(q_3) + 1.0*cos(q_1)*cos(q_3)*sin(q_2))*(0.0016*cos(q_1)*(1.0*sin(q_1)*sin(q_2)*sin(q_3) - 1.0*cos(q_2)*cos(q_3)*sin(q_1)) + 0.0016*sin(q_1)*(cos(q_1)*cos(q_2)*cos(q_3) - 1.0*cos(q_1)*sin(q_2)*sin(q_3)))) - 1.0*(0.2723*cos(q_2)*cos(q_3) - 0.2723*sin(q_2)*sin(q_3))*(0.6195*cos(q_2)*sin(q_3) + 0.6195*cos(q_3)*sin(q_2)) - 1.0*(0.2723*cos(q_2)*sin(q_3) + 0.2723*cos(q_3)*sin(q_2))*(0.6195*cos(q_2)*cos(q_3) - 0.6195*sin(q_2)*sin(q_3)) + 4.55*cos(q_1)^2*(0.2723*cos(q_2)*cos(q_3) - 0.2723*sin(q_2)*sin(q_3))*(0.2723*cos(q_2)*sin(q_3) + 0.2723*cos(q_3)*sin(q_2)) + 4.55*sin(q_1)^2*(0.2723*cos(q_2)*cos(q_3) - 0.2723*sin(q_2)*sin(q_3))*(0.2723*cos(q_2)*sin(q_3) + 0.2723*cos(q_3)*sin(q_2)))];




%Gravity
G = [                                                                                             0;
1.784*g*cos(q_2) - 2.275*g*(0.2723*sin(q_2)*sin(q_3) - 1.0*cos(q_2)*(0.2723*cos(q_3) + 0.425));
                                 2.275*g*(0.2723*cos(q_2)*cos(q_3) - 0.2723*sin(q_2)*sin(q_3))];
